simulink model "TailSitter_waypoints_continuous"  (R2018b)
settings: Solver=VariableStepAuto  StartTime=0.0  StopTime=400  RelTol=1e-3
values from neighbouring files (symbols this model uses):
  p =     [ds.mat]    (also in vxs.mat)
undefined symbols (not defined in the file or in its folder): quatnormalize
libraries: aerolibutil x18, simulink x6, sharedutil x3, vrlib x2, simulink_extras x2, sharedtransform x1
(part 2 of 4)

== matlab function TailSitter_waypoints_continuous/Torque_FL ==
  data: u_omegaL output; u_omegaR output; u_deltaL output; u_deltaR output; tao input; states input; u_jointT input; p parameter
function [u_omegaL,u_omegaR, u_deltaL,u_deltaR]  = FL_torques(tao, states, u_jointT, p)


wxr = tao(1); % I wonder if this comversion from omega to tao is right? Depends on Emil Fresk implementation
wyr = tao(2);
wzr = tao(3);
v = states(1:3);
vx = v(1);
vy = v(2);
vz = v(3);
w = states(4:6);
wx = w(1);
wy = w(2);
wz = w(3);
q = states(7:10); % Possibly not needed?
q0=q(1);
q1=q(2);
q2=q(3);
q3=(4);
deltaL = states(11);
deltaR = states(12);
omegaL = states(13);
omegaR = states(14);

% init output vector
u_deltaL = 0;
u_deltaR = 0;
u_omegaL = 0;
u_omegaR = 0;

% If you know of a better way (not counting modifying the code below to use
% p.x notation, plese feel welcome to tell me.
%P = struct2cell(p);
%Pn = fieldnames(p);
%for i=1:numel(P)
%    eval(Pn{i}+"="+string(P{i})+";")
%end
Ts=p.Ts;
m=p.m;
Ix=p.Ix;
Iy=p.Iy;
Iz=p.Iz;
I=p.I;
g=p.g;
rho=p.rho;
propd=p.propd;
K_T=p.K_T;
K_v=p.K_v;
b_w=p.b_w;
Sa=p.Sa;
Saw=p.Saw;
CLdelta=p.CLdelta;
CDdelta=p.CDdelta;
SW=p.SW;
Sw_w=p.Sw_w;
Sw=p.Sw;
b=p.b;
Cmyl=p.Cmyl;
Cwy=p.Cwy;
yf=p.yf;
yt=p.yt;
xW=p.xW;
xf=p.xf;
xac=p.xac;
zW=p.zW;
yw=p.yw;
yW=p.yW;
yWE=p.yWE;
yWEE=p.yWEE;
K_omegaL=p.K_omegaL;
K_omegaR=p.K_omegaR;
K_deltaL=p.K_deltaL;
K_deltaR=p.K_deltaR;
CL_A=p.CL_A;
CL_B=p.CL_B;
CL_C=p.CL_C;
CD_A=p.CD_A;
CD_B=p.CD_B;
CD_C=p.CD_C;
CLB_A=p.CLB_A;
CLB_B=p.CLB_B;
CDB_A=p.CDB_A;
CDB_B=p.CDB_B;
% The constants below are for the polynomial approximations.
% I am lookin into a way of auto-generating them in a struct or something.
a11=p.a11;
a12=p.a12;
a13=p.a13;
a21=p.a21;
a22=p.a22;
a23=p.a23;
a31=p.a31;
a32=p.a32;
a33=p.a33;
a41=p.a41;
a42=p.a42;
a43=p.a43;
b11=p.b11;
b12=p.b12;
b13=p.b13;
b14=p.b14;
b21=p.b21;
b22=p.b22;
b23=p.b23;
b24=p.b24;
b31=p.b31;
b32=p.b32;
b33=p.b33;
b34=p.b34;
c11=p.c11;
c12=p.c12;
c13=p.c13;
c14=p.c14;
c21=p.c21;
c22=p.c22;
c23=p.c23;
c24=p.c24;
c31=p.c31;
c32=p.c32;
c33=p.c33;
c34=p.c34;
c41=p.c41;
c42=p.c42;
c43=p.c43;
c44=p.c44;
% Assuming we made correct choices here it should suffice with this:
%u = [u_deltaA u_jointA u_deltaT]';


% Hey, anyone reading this? Code below is auto-generated because the
% F.L. was just too much of a headache to do
% manyally, so I wrote a script for it.
wn = p.wn;
u_ref =[ ...
                                                                                                                                                                                                                                                                                                                                                                                                                                                                                                                                                                                                                                                                                                                                                                                                                                                                                                                                                                                                                                                                                                                                                                                                                                                                                                                                                                                                                                                                                                                                                                                                                                                                                                                                                                                                                                                                                                                                                                                                                                                                                                                                                                                                                                                                                                                                                                                                                                                                                                                                                                                                                                                                                                                                                                                                                                                                                                                                                                                                                                                                                                                                                                                                                                                                                                                                                                                                                                                                                                                                                                                                                                                                                                                                                                                                                                                                                                                                                                                                                                                                                                                                                                                                                                                                                                                                                                                                                                                                                                                                                                                                                                                                                                                                                                                                                                                                                                                                                                                                                                                                                                                                                                                                                                                                                                                                                                                                                                                                                                                                                                                                                                                                                                                                                                                                                                                                                                                                                                                                                                                                                                                                                                                                                                                                                                                                                                                                                                                                                                                                                                                                                                                                                                                                                                                                                                                                                                                                                                                                                                                                                                                                                                                                                                                                                                                                                                                                                                                                                                                                                                                                                                                                                                                                                                                                                                                                                                                                                                                                                                                                                                                                                                                                                                                                                                                                                                                                                                                                                                                                                                                                                                                                                                                                                                                                                                                                                                                                                                                                                                                                                                                                                                                                                                                                                                                                                                                                                                                                                                                                                                                                                                                                                                                                                                                                                                                                                                                                                                                                                                                                                                                                                                                                                                                                                                                                                                                                                                                                                                                                                                                                                                                                                                                                                                                                                                                                                                                                                                                                                                                                                                                                                                                                                                                                                                                                                                                                                                                                                                                                                                                                                                                                                                                                                                                                                                                                                                                                                                                                                                                                                                                                                                                                                                                                                                                                                                                                                                                                                                                                                                                                                                                                                                                                                                                                                                                                                                                                                                 (4.24e-22*(3.02e112*omegaL^4*wn*abs(omegaL) - 7.01e117*omegaR^3*atan2(1.0*vz, vx) + 1.2e116*omegaL^2*atan2(1.0*vz, vx)*abs(omegaL) - 1.2e116*omegaL^2*atan2(1.0*vz, vx)*abs(omegaR) - 1.2e116*omegaR^2*atan2(1.0*vz, vx)*abs(omegaL) + 1.2e116*omegaR^2*atan2(1.0*vz, vx)*abs(omegaR) + 1.2e116*omegaL^3*atan2(1.0*vz, vx)*sign(omegaL) + 1.2e116*omegaR^3*atan2(1.0*vz, vx)*sign(omegaR) - 4.77e117*omegaL^3*atan2(1.0*vz, vx) + 3.02e112*omegaL^4*wn*abs(omegaR) - 3.02e112*omegaR^4*wn*abs(omegaL) - 3.02e112*omegaR^4*wn*abs(omegaR) + 5.89e117*omegaL^3*wn^2*wx + 5.89e117*omegaR^3*wn^2*wx + 5.89e117*omegaL^3*wn^2*wxr + 5.89e117*omegaR^3*wn^2*wxr - 1.12e117*omegaL^3*wn^2*wy + 1.12e117*omegaR^3*wn^2*wy - 1.12e117*omegaL^3*wn^2*wyr + 1.12e117*omegaR^3*wn^2*wyr - 3.02e112*omegaL^5*wn*sign(omegaL) + 3.02e112*omegaR^5*wn*sign(omegaR) - 7.01e117*omegaL*omegaR^2*atan2(1.0*vz, vx) - 4.77e117*omegaL^2*omegaR*atan2(1.0*vz, vx) - 1.2e116*omegaL^2*wn^2*wz*abs(omegaL) + 1.2e116*omegaL^2*wn^2*wz*abs(omegaR) + 1.2e116*omegaR^2*wn^2*wz*abs(omegaL) - 1.2e116*omegaR^2*wn^2*wz*abs(omegaR) - 1.2e116*omegaL^2*wn^2*wzr*abs(omegaL) + 1.2e116*omegaL^2*wn^2*wzr*abs(omegaR) + 1.2e116*omegaR^2*wn^2*wzr*abs(omegaL) - 1.2e116*omegaR^2*wn^2*wzr*abs(omegaR) - 5.43e117*deltaL*omegaL*omegaR^2*atan2(1.0*vz, vx) - 5.43e117*deltaR*omegaL^2*omegaR*atan2(1.0*vz, vx) + 6.04e112*omegaL^3*omegaR^2*wn*sign(omegaL) - 6.04e112*omegaL^2*omegaR^3*wn*sign(omegaR) - 1.2e116*omegaL^3*wn^2*wz*sign(omegaL) - 1.2e116*omegaR^3*wn^2*wz*sign(omegaR) - 1.2e116*omegaL^3*wn^2*wzr*sign(omegaL) - 1.2e116*omegaR^3*wn^2*wzr*sign(omegaR) - 1.37e114*deltaL*omegaL*omegaR^4*wn + 1.37e114*deltaR*omegaL^4*omegaR*wn + 1.68e119*a11*omegaL^3*wn*wx + 1.68e119*a11*omegaR^3*wn*wx + 1.68e119*b11*omegaL^3*wn*wz + 1.68e119*b11*omegaR^3*wn*wz - 2.89e116*omegaL^3*vx*wn*(vx^2 + vy^2)^(1/2) + 2.89e116*omegaR^3*vx*wn*(vx^2 + vy^2)^(1/2) + 1.16e116*omegaL^3*vx*wn*(vx^2 + vz^2)^(1/2) - 1.71e116*omegaL^3*vy*wn*(vx^2 + vy^2)^(1/2) - 1.16e116*omegaR^3*vx*wn*(vx^2 + vz^2)^(1/2) - 1.71e116*omegaR^3*vy*wn*(vx^2 + vy^2)^(1/2) + 1.19e117*omegaL^3*vz*wn*(vx^2 + vz^2)^(1/2) - 1.19e117*omegaR^3*vz*wn*(vx^2 + vz^2)^(1/2) + 5.8e118*omegaL^3*wn*wy*(vx^2 + vz^2)^(1/2) - 5.8e118*omegaR^3*wn*wy*(vx^2 + vz^2)^(1/2) - 1.2e116*omegaL*omegaR^2*atan2(1.0*vz, vx)*sign(omegaL) - 1.2e116*omegaL^2*omegaR*atan2(1.0*vz, vx)*sign(omegaR) - 1.37e114*deltaL*omegaL^2*omegaR^3*wn + 1.37e114*deltaR*omegaL^3*omegaR^2*wn - 1.02e121*omegaL*vx^2*atan2(1.0*vz, vx)*sign(vx) - 1.02e121*omegaR*vx^2*atan2(1.0*vz, vx)*sign(vx) - 1.02e121*omegaL*vy^2*atan2(1.0*vz, vx)*sign(vx) - 1.02e121*omegaR*vy^2*atan2(1.0*vz, vx)*sign(vx) - 1.02e121*omegaL*vz^2*atan2(1.0*vz, vx)*sign(vx) - 1.02e121*omegaR*vz^2*atan2(1.0*vz, vx)*sign(vx) - 6.04e112*omegaL*omegaR^3*wn*abs(omegaL) + 6.04e112*omegaL^3*omegaR*wn*abs(omegaL) - 6.04e112*omegaL*omegaR^3*wn*abs(omegaR) + 6.04e112*omegaL^3*omegaR*wn*abs(omegaR) + 5.89e117*omegaL*omegaR^2*wn^2*wx + 5.89e117*omegaL^2*omegaR*wn^2*wx + 5.89e117*omegaL*omegaR^2*wn^2*wxr + 5.89e117*omegaL^2*omegaR*wn^2*wxr + 1.12e117*omegaL*omegaR^2*wn^2*wy - 1.12e117*omegaL^2*omegaR*wn^2*wy + 1.12e117*omegaL*omegaR^2*wn^2*wyr - 1.12e117*omegaL^2*omegaR*wn^2*wyr - 3.02e112*omegaL*omegaR^4*wn*sign(omegaL) + 3.02e112*omegaL^4*omegaR*wn*sign(omegaR) - 4.72e120*deltaL*omegaL*vx^2*atan2(1.0*vz, vx)*sign(vx) - 4.72e120*deltaR*omegaR*vx^2*atan2(1.0*vz, vx)*sign(vx) - 4.72e120*deltaL*omegaL*vy^2*atan2(1.0*vz, vx)*sign(vx) - 4.72e120*deltaR*omegaR*vy^2*atan2(1.0*vz, vx)*sign(vx) - 4.72e120*deltaL*omegaL*vz^2*atan2(1.0*vz, vx)*sign(vx) - 4.72e120*deltaR*omegaR*vz^2*atan2(1.0*vz, vx)*sign(vx) + 5.43e117*deltaL*omegaL*omegaR^2*wn^2*wz + 5.43e117*deltaR*omegaL^2*omegaR*wn^2*wz + 5.43e117*deltaL*omegaL*omegaR^2*wn^2*wzr + 5.43e117*deltaR*omegaL^2*omegaR*wn^2*wzr - 3.0e117*c11*omegaL^2*wn*wz*abs(omegaL) + 3.0e117*c11*omegaL^2*wn*wz*abs(omegaR) + 3.0e117*c11*omegaR^2*wn*wz*abs(omegaL) - 3.0e117*c11*omegaR^2*wn*wz*abs(omegaR) + 1.68e119*a31*omegaL^3*vx^2*wn*wx + 1.68e119*a31*omegaR^3*vx^2*wn*wx + 1.68e119*a41*omegaL^3*vx^3*wn*wx + 1.68e119*a41*omegaR^3*vx^3*wn*wx + 1.68e119*a13*omegaL^3*vz^2*wn*wx + 1.68e119*a13*omegaR^3*vz^2*wn*wx + 1.68e119*b31*omegaL^3*vx^2*wn*wz + 1.68e119*b31*omegaR^3*vx^2*wn*wz + 1.68e119*b13*omegaL^3*vz^2*wn*wz + 1.68e119*b14*omegaL^3*vz^3*wn*wz + 1.68e119*b13*omegaR^3*vz^2*wn*wz + 1.68e119*b14*omegaR^3*vz^3*wn*wz - 2.75e115*omegaL^2*vy*wn*abs(omegaL)*(vx^2 + vy^2)^(1/2) + 2.75e115*omegaL^2*vy*wn*abs(omegaR)*(vx^2 + vy^2)^(1/2) + 2.75e115*omegaR^2*vy*wn*abs(omegaL)*(vx^2 + vy^2)^(1/2) - 2.75e115*omegaR^2*vy*wn*abs(omegaR)*(vx^2 + vy^2)^(1/2) - 3.0e117*c11*omegaL^3*wn*wz*sign(omegaL) - 3.0e117*c11*omegaR^3*wn*wz*sign(omegaR) - 2.75e115*omegaL^3*vy*wn*sign(omegaL)*(vx^2 + vy^2)^(1/2) - 2.75e115*omegaR^3*vy*wn*sign(omegaR)*(vx^2 + vy^2)^(1/2) - 2.98e119*omegaL*vy^3*wn*sign(vx)*(vx^2 + vy^2)^(1/2) - 2.98e119*omegaR*vy^3*wn*sign(vx)*(vx^2 + vy^2)^(1/2) - 1.03e120*deltaL*omegaL*vx^4*wn*sign(vx)^2 - 1.19e117*deltaL*omegaR^3*vx^2*wn*sign(vx) + 1.19e117*deltaR*omegaL^3*vx^2*wn*sign(vx) - 1.03e120*deltaL*omegaR*vx^4*wn*sign(vx)^2 + 1.03e120*deltaR*omegaL*vx^4*wn*sign(vx)^2 + 1.03e120*deltaR*omegaR*vx^4*wn*sign(vx)^2 - 1.03e120*deltaL*omegaL*vy^4*wn*sign(vx)^2 - 1.19e117*deltaL*omegaR^3*vy^2*wn*sign(vx) + 1.19e117*deltaR*omegaL^3*vy^2*wn*sign(vx) - 1.03e120*deltaL*omegaR*vy^4*wn*sign(vx)^2 + 1.03e120*deltaR*omegaL*vy^4*wn*sign(vx)^2 + 1.03e120*deltaR*omegaR*vy^4*wn*sign(vx)^2 - 1.03e120*deltaL*omegaL*vz^4*wn*sign(vx)^2 - 1.19e117*deltaL*omegaR^3*vz^2*wn*sign(vx) + 1.19e117*deltaR*omegaL^3*vz^2*wn*sign(vx) - 1.03e120*deltaL*omegaR*vz^4*wn*sign(vx)^2 + 1.03e120*deltaR*omegaL*vz^4*wn*sign(vx)^2 + 1.03e120*deltaR*omegaR*vz^4*wn*sign(vx)^2 + 1.2e116*omegaL*omegaR^2*wn^2*wz*sign(omegaL) + 1.2e116*omegaL^2*omegaR*wn^2*wz*sign(omegaR) + 1.2e116*omegaL*omegaR^2*wn^2*wzr*sign(omegaL) + 1.2e116*omegaL^2*omegaR*wn^2*wzr*sign(omegaR) + 2.89e116*omegaL^3*vx*wn*cos(2.0*atan2(1.0*vy, vx))*(vx^2 + vy^2)^(1/2) - 2.89e116*omegaR^3*vx*wn*cos(2.0*atan2(1.0*vy, vx))*(vx^2 + vy^2)^(1/2) + 1.71e116*omegaL^3*vy*wn*cos(2.0*atan2(1.0*vy, vx))*(vx^2 + vy^2)^(1/2) + 1.71e116*omegaR^3*vy*wn*cos(2.0*atan2(1.0*vy, vx))*(vx^2 + vy^2)^(1/2) - 1.16e117*omegaL^3*vz*wn*cos(2.0*atan2(1.0*vz, vx))*(vx^2 + vz^2)^(1/2) + 1.16e117*omegaR^3*vz*wn*cos(2.0*atan2(1.0*vz, vx))*(vx^2 + vz^2)^(1/2) + 1.02e121*omegaL*vx^2*wn^2*wx*sign(vx) + 1.02e121*omegaR*vx^2*wn^2*wx*sign(vx) + 1.02e121*omegaL*vx^2*wn^2*wxr*sign(vx) + 1.02e121*omegaR*vx^2*wn^2*wxr*sign(vx) + 1.02e121*omegaL*vy^2*wn^2*wx*sign(vx) + 1.02e121*omegaR*vy^2*wn^2*wx*sign(vx) + 1.02e121*omegaL*vy^2*wn^2*wxr*sign(vx) + 1.02e121*omegaR*vy^2*wn^2*wxr*sign(vx) + 1.02e121*omegaL*vz^2*wn^2*wx*sign(vx) + 1.02e121*omegaR*vz^2*wn^2*wx*sign(vx) + 1.02e121*omegaL*vz^2*wn^2*wxr*sign(vx) + 1.02e121*omegaR*vz^2*wn^2*wxr*sign(vx) - 1.03e116*omegaL^3*vx*wn*sin(2.0*atan2(1.0*vy, vx))*(vx^2 + vy^2)^(1/2) - 1.03e116*omegaR^3*vx*wn*sin(2.0*atan2(1.0*vy, vx))*(vx^2 + vy^2)^(1/2) + 1.73e116*omegaL^3*vy*wn*sin(2.0*atan2(1.0*vy, vx))*(vx^2 + vy^2)^(1/2) - 1.73e116*omegaR^3*vy*wn*sin(2.0*atan2(1.0*vy, vx))*(vx^2 + vy^2)^(1/2) + 6.96e116*omegaL^3*vx*wn*sin(2.0*atan2(1.0*vz, vx))*(vx^2 + vz^2)^(1/2) - 6.96e116*omegaR^3*vx*wn*sin(2.0*atan2(1.0*vz, vx))*(vx^2 + vz^2)^(1/2) + 1.68e119*a11*omegaL*omegaR^2*wn*wx + 1.68e119*a11*omegaL^2*omegaR*wn*wx + 1.68e119*b11*omegaL*omegaR^2*wn*wz + 1.68e119*b11*omegaL^2*omegaR*wn*wz + 1.68e119*a21*omegaL^3*vx*wn*wx + 1.68e119*a21*omegaR^3*vx*wn*wx + 1.68e119*a12*omegaL^3*vz*wn*wx + 1.68e119*a12*omegaR^3*vz*wn*wx + 1.68e119*b21*omegaL^3*vx*wn*wz + 1.68e119*b21*omegaR^3*vx*wn*wz + 1.68e119*b12*omegaL^3*vz*wn*wz + 1.68e119*b12*omegaR^3*vz*wn*wz + 2.89e116*omegaL*omegaR^2*vx*wn*(vx^2 + vy^2)^(1/2) - 2.89e116*omegaL^2*omegaR*vx*wn*(vx^2 + vy^2)^(1/2) - 1.16e116*omegaL*omegaR^2*vx*wn*(vx^2 + vz^2)^(1/2) - 1.71e116*omegaL*omegaR^2*vy*wn*(vx^2 + vy^2)^(1/2) + 1.16e116*omegaL^2*omegaR*vx*wn*(vx^2 + vz^2)^(1/2) - 1.71e116*omegaL^2*omegaR*vy*wn*(vx^2 + vy^2)^(1/2) - 1.19e117*omegaL*omegaR^2*vz*wn*(vx^2 + vz^2)^(1/2) + 1.19e117*omegaL^2*omegaR*vz*wn*(vx^2 + vz^2)^(1/2) - 5.8e118*omegaL*omegaR^2*wn*wy*(vx^2 + vz^2)^(1/2) + 5.8e118*omegaL^2*omegaR*wn*wy*(vx^2 + vz^2)^(1/2) - 3.0e117*c31*omegaL^2*vx^2*wn*wz*abs(omegaL) + 3.0e117*c31*omegaL^2*vx^2*wn*wz*abs(omegaR) + 3.0e117*c31*omegaR^2*vx^2*wn*wz*abs(omegaL) - 3.0e117*c41*omegaL^2*vx^3*wn*wz*abs(omegaL) - 3.0e117*c31*omegaR^2*vx^2*wn*wz*abs(omegaR) + 3.0e117*c41*omegaL^2*vx^3*wn*wz*abs(omegaR) + 3.0e117*c41*omegaR^2*vx^3*wn*wz*abs(omegaL) - 3.0e117*c41*omegaR^2*vx^3*wn*wz*abs(omegaR) - 3.0e117*c13*omegaL^2*vz^2*wn*wz*abs(omegaL) - 3.0e117*c14*omegaL^2*vz^3*wn*wz*abs(omegaL) + 3.0e117*c13*omegaL^2*vz^2*wn*wz*abs(omegaR) + 3.0e117*c13*omegaR^2*vz^2*wn*wz*abs(omegaL) + 3.0e117*c14*omegaL^2*vz^3*wn*wz*abs(omegaR) + 3.0e117*c14*omegaR^2*vz^3*wn*wz*abs(omegaL) - 3.0e117*c13*omegaR^2*vz^2*wn*wz*abs(omegaR) - 3.0e117*c14*omegaR^2*vz^3*wn*wz*abs(omegaR) + 1.68e119*a33*omegaL^3*vx^2*vz^2*wn*wx + 1.68e119*a33*omegaR^3*vx^2*vz^2*wn*wx + 1.68e119*a43*omegaL^3*vx^3*vz^2*wn*wx + 1.68e119*a43*omegaR^3*vx^3*vz^2*wn*wx + 1.68e119*b33*omegaL^3*vx^2*vz^2*wn*wz + 1.68e119*b34*omegaL^3*vx^2*vz^3*wn*wz + 1.68e119*b33*omegaR^3*vx^2*vz^2*wn*wz + 1.68e119*b34*omegaR^3*vx^2*vz^3*wn*wz - 3.0e117*c31*omegaL^3*vx^2*wn*wz*sign(omegaL) - 3.0e117*c41*omegaL^3*vx^3*wn*wz*sign(omegaL) - 3.0e117*c31*omegaR^3*vx^2*wn*wz*sign(omegaR) - 3.0e117*c41*omegaR^3*vx^3*wn*wz*sign(omegaR) - 3.0e117*c13*omegaL^3*vz^2*wn*wz*sign(omegaL) - 3.0e117*c14*omegaL^3*vz^3*wn*wz*sign(omegaL) - 3.0e117*c13*omegaR^3*vz^2*wn*wz*sign(omegaR) - 3.0e117*c14*omegaR^3*vz^3*wn*wz*sign(omegaR) - 2.37e117*deltaL*omegaL*omegaR^2*vx^2*wn*sign(vx) - 1.19e117*deltaL*omegaL^2*omegaR*vx^2*wn*sign(vx) + 1.19e117*deltaR*omegaL*omegaR^2*vx^2*wn*sign(vx) + 2.37e117*deltaR*omegaL^2*omegaR*vx^2*wn*sign(vx) - 2.37e117*deltaL*omegaL*omegaR^2*vy^2*wn*sign(vx) - 1.19e117*deltaL*omegaL^2*omegaR*vy^2*wn*sign(vx) + 1.19e117*deltaR*omegaL*omegaR^2*vy^2*wn*sign(vx) + 2.37e117*deltaR*omegaL^2*omegaR*vy^2*wn*sign(vx) - 2.37e117*deltaL*omegaL*omegaR^2*vz^2*wn*sign(vx) - 1.19e117*deltaL*omegaL^2*omegaR*vz^2*wn*sign(vx) + 1.19e117*deltaR*omegaL*omegaR^2*vz^2*wn*sign(vx) + 2.37e117*deltaR*omegaL^2*omegaR*vz^2*wn*sign(vx) + 4.72e120*deltaL*omegaL*vx^2*wn^2*wz*sign(vx) + 4.72e120*deltaR*omegaR*vx^2*wn^2*wz*sign(vx) + 4.72e120*deltaL*omegaL*vx^2*wn^2*wzr*sign(vx) + 4.72e120*deltaR*omegaR*vx^2*wn^2*wzr*sign(vx) + 4.72e120*deltaL*omegaL*vy^2*wn^2*wz*sign(vx) + 4.72e120*deltaR*omegaR*vy^2*wn^2*wz*sign(vx) + 4.72e120*deltaL*omegaL*vy^2*wn^2*wzr*sign(vx) + 4.72e120*deltaR*omegaR*vy^2*wn^2*wzr*sign(vx) + 4.72e120*deltaL*omegaL*vz^2*wn^2*wz*sign(vx) + 4.72e120*deltaR*omegaR*vz^2*wn^2*wz*sign(vx) + 4.72e120*deltaL*omegaL*vz^2*wn^2*wzr*sign(vx) + 4.72e120*deltaR*omegaR*vz^2*wn^2*wzr*sign(vx) - 2.89e116*omegaL*omegaR^2*vx*wn*cos(2.0*atan2(1.0*vy, vx))*(vx^2 + vy^2)^(1/2) + 2.89e116*omegaL^2*omegaR*vx*wn*cos(2.0*atan2(1.0*vy, vx))*(vx^2 + vy^2)^(1/2) + 1.71e116*omegaL*omegaR^2*vy*wn*cos(2.0*atan2(1.0*vy, vx))*(vx^2 + vy^2)^(1/2) + 1.71e116*omegaL^2*omegaR*vy*wn*cos(2.0*atan2(1.0*vy, vx))*(vx^2 + vy^2)^(1/2) + 1.16e117*omegaL*omegaR^2*vz*wn*cos(2.0*atan2(1.0*vz, vx))*(vx^2 + vz^2)^(1/2) - 1.16e117*omegaL^2*omegaR*vz*wn*cos(2.0*atan2(1.0*vz, vx))*(vx^2 + vz^2)^(1/2) + 1.36e119*c11*deltaL*omegaL*omegaR^2*wn*wz + 1.36e119*c11*deltaR*omegaL^2*omegaR*wn*wz - 1.03e116*omegaL*omegaR^2*vx*wn*sin(2.0*atan2(1.0*vy, vx))*(vx^2 + vy^2)^(1/2) - 1.03e116*omegaL^2*omegaR*vx*wn*sin(2.0*atan2(1.0*vy, vx))*(vx^2 + vy^2)^(1/2) - 1.73e116*omegaL*omegaR^2*vy*wn*sin(2.0*atan2(1.0*vy, vx))*(vx^2 + vy^2)^(1/2) + 1.73e116*omegaL^2*omegaR*vy*wn*sin(2.0*atan2(1.0*vy, vx))*(vx^2 + vy^2)^(1/2) - 6.96e116*omegaL*omegaR^2*vx*wn*sin(2.0*atan2(1.0*vz, vx))*(vx^2 + vz^2)^(1/2) + 6.96e116*omegaL^2*omegaR*vx*wn*sin(2.0*atan2(1.0*vz, vx))*(vx^2 + vz^2)^(1/2) + 1.25e117*deltaL*omegaL*omegaR^2*vy*wn*(vx^2 + vy^2)^(1/2) + 1.25e117*deltaR*omegaL^2*omegaR*vy*wn*(vx^2 + vy^2)^(1/2) + 1.68e119*a21*omegaL*omegaR^2*vx*wn*wx + 1.68e119*a21*omegaL^2*omegaR*vx*wn*wx + 1.68e119*a12*omegaL*omegaR^2*vz*wn*wx + 1.68e119*a12*omegaL^2*omegaR*vz*wn*wx + 1.68e119*b21*omegaL*omegaR^2*vx*wn*wz + 1.68e119*b21*omegaL^2*omegaR*vx*wn*wz + 1.68e119*b12*omegaL*omegaR^2*vz*wn*wz + 1.68e119*b12*omegaL^2*omegaR*vz*wn*wz + 1.68e119*a22*omegaL^3*vx*vz*wn*wx + 1.68e119*a22*omegaR^3*vx*vz*wn*wx + 1.68e119*b22*omegaL^3*vx*vz*wn*wz + 1.68e119*b22*omegaR^3*vx*vz*wn*wz - 2.06e120*deltaL*omegaL*vx^2*vy^2*wn*sign(vx)^2 - 2.06e120*deltaL*omegaR*vx^2*vy^2*wn*sign(vx)^2 + 2.06e120*deltaR*omegaL*vx^2*vy^2*wn*sign(vx)^2 + 2.06e120*deltaR*omegaR*vx^2*vy^2*wn*sign(vx)^2 - 2.06e120*deltaL*omegaL*vx^2*vz^2*wn*sign(vx)^2 - 2.06e120*deltaL*omegaR*vx^2*vz^2*wn*sign(vx)^2 + 2.06e120*deltaR*omegaL*vx^2*vz^2*wn*sign(vx)^2 + 2.06e120*deltaR*omegaR*vx^2*vz^2*wn*sign(vx)^2 - 2.06e120*deltaL*omegaL*vy^2*vz^2*wn*sign(vx)^2 - 2.06e120*deltaL*omegaR*vy^2*vz^2*wn*sign(vx)^2 + 2.06e120*deltaR*omegaL*vy^2*vz^2*wn*sign(vx)^2 + 2.06e120*deltaR*omegaR*vy^2*vz^2*wn*sign(vx)^2 + 2.75e115*omegaL^2*vy*wn*cos(2.0*atan2(1.0*vy, vx))*abs(omegaL)*(vx^2 + vy^2)^(1/2) - 2.75e115*omegaL^2*vy*wn*cos(2.0*atan2(1.0*vy, vx))*abs(omegaR)*(vx^2 + vy^2)^(1/2) - 2.75e115*omegaR^2*vy*wn*cos(2.0*atan2(1.0*vy, vx))*abs(omegaL)*(vx^2 + vy^2)^(1/2) + 2.75e115*omegaR^2*vy*wn*cos(2.0*atan2(1.0*vy, vx))*abs(omegaR)*(vx^2 + vy^2)^(1/2) - 1.65e115*omegaL^2*vx*wn*sin(2.0*atan2(1.0*vy, vx))*abs(omegaL)*(vx^2 + vy^2)^(1/2) + 1.65e115*omegaL^2*vx*wn*sin(2.0*atan2(1.0*vy, vx))*abs(omegaR)*(vx^2 + vy^2)^(1/2) + 1.65e115*omegaR^2*vx*wn*sin(2.0*atan2(1.0*vy, vx))*abs(omegaL)*(vx^2 + vy^2)^(1/2) - 1.65e115*omegaR^2*vx*wn*sin(2.0*atan2(1.0*vy, vx))*abs(omegaR)*(vx^2 + vy^2)^(1/2) + 2.75e115*omegaL^3*vy*wn*cos(2.0*atan2(1.0*vy, vx))*sign(omegaL)*(vx^2 + vy^2)^(1/2) + 2.75e115*omegaR^3*vy*wn*cos(2.0*atan2(1.0*vy, vx))*sign(omegaR)*(vx^2 + vy^2)^(1/2) + 2.98e119*omegaL*vy^3*wn*cos(2.0*atan2(1.0*vy, vx))*sign(vx)*(vx^2 + vy^2)^(1/2) + 2.98e119*omegaR*vy^3*wn*cos(2.0*atan2(1.0*vy, vx))*sign(vx)*(vx^2 + vy^2)^(1/2) + 1.68e119*a31*omegaL*omegaR^2*vx^2*wn*wx + 1.68e119*a31*omegaL^2*omegaR*vx^2*wn*wx + 1.68e119*a41*omegaL*omegaR^2*vx^3*wn*wx + 1.68e119*a41*omegaL^2*omegaR*vx^3*wn*wx + 1.68e119*a13*omegaL*omegaR^2*vz^2*wn*wx + 1.68e119*a13*omegaL^2*omegaR*vz^2*wn*wx + 1.68e119*b31*omegaL*omegaR^2*vx^2*wn*wz + 1.68e119*b31*omegaL^2*omegaR*vx^2*wn*wz + 1.68e119*b13*omegaL*omegaR^2*vz^2*wn*wz + 1.68e119*b13*omegaL^2*omegaR*vz^2*wn*wz + 1.68e119*b14*omegaL*omegaR^2*vz^3*wn*wz + 1.68e119*b14*omegaL^2*omegaR*vz^3*wn*wz - 3.0e117*c21*omegaL^2*vx*wn*wz*abs(omegaL) + 3.0e117*c21*omegaL^2*vx*wn*wz*abs(omegaR) + 3.0e117*c21*omegaR^2*vx*wn*wz*abs(omegaL) - 3.0e117*c21*omegaR^2*vx*wn*wz*abs(omegaR) - 3.0e117*c12*omegaL^2*vz*wn*wz*abs(omegaL) + 3.0e117*c12*omegaL^2*vz*wn*wz*abs(omegaR) + 3.0e117*c12*omegaR^2*vz*wn*wz*abs(omegaL) - 3.0e117*c12*omegaR^2*vz*wn*wz*abs(omegaR) - 1.65e115*omegaL^3*vx*wn*sin(2.0*atan2(1.0*vy, vx))*sign(omegaL)*(vx^2 + vy^2)^(1/2) - 1.65e115*omegaR^3*vx*wn*sin(2.0*atan2(1.0*vy, vx))*sign(omegaR)*(vx^2 + vy^2)^(1/2) + 1.68e119*a23*omegaL^3*vx*vz^2*wn*wx + 1.68e119*a23*omegaR^3*vx*vz^2*wn*wx + 1.68e119*a32*omegaL^3*vx^2*vz*wn*wx + 1.68e119*a32*omegaR^3*vx^2*vz*wn*wx + 1.68e119*a42*omegaL^3*vx^3*vz*wn*wx + 1.68e119*a42*omegaR^3*vx^3*vz*wn*wx + 1.68e119*b23*omegaL^3*vx*vz^2*wn*wz + 1.68e119*b24*omegaL^3*vx*vz^3*wn*wz + 1.68e119*b23*omegaR^3*vx*vz^2*wn*wz + 1.68e119*b24*omegaR^3*vx*vz^3*wn*wz + 1.68e119*b32*omegaL^3*vx^2*vz*wn*wz + 1.68e119*b32*omegaR^3*vx^2*vz*wn*wz - 1.79e119*omegaL*vx^3*wn*sin(2.0*atan2(1.0*vy, vx))*sign(vx)*(vx^2 + vy^2)^(1/2) - 1.79e119*omegaR*vx^3*wn*sin(2.0*atan2(1.0*vy, vx))*sign(vx)*(vx^2 + vy^2)^(1/2) + 3.0e117*c11*omegaL*omegaR^2*wn*wz*sign(omegaL) + 3.0e117*c11*omegaL^2*omegaR*wn*wz*sign(omegaR) + 1.08e120*deltaL*omegaL*vy^3*wn*sign(vx)*(vx^2 + vy^2)^(1/2) + 1.08e120*deltaR*omegaR*vy^3*wn*sign(vx)*(vx^2 + vy^2)^(1/2) + 2.75e115*omegaL*omegaR^2*vy*wn*sign(omegaL)*(vx^2 + vy^2)^(1/2) + 2.75e115*omegaL^2*omegaR*vy*wn*sign(omegaR)*(vx^2 + vy^2)^(1/2) - 3.0e117*c21*omegaL^3*vx*wn*wz*sign(omegaL) - 3.0e117*c21*omegaR^3*vx*wn*wz*sign(omegaR) - 3.0e117*c12*omegaL^3*vz*wn*wz*sign(omegaL) - 3.0e117*c12*omegaR^3*vz*wn*wz*sign(omegaR) + 2.92e122*a11*omegaL*vx^2*wn*wx*sign(vx) + 2.92e122*a11*omegaR*vx^2*wn*wx*sign(vx) + 2.92e122*a21*omegaL*vx^3*wn*wx*sign(vx) + 2.92e122*a21*omegaR*vx^3*wn*wx*sign(vx) + 2.92e122*a31*omegaL*vx^4*wn*wx*sign(vx) + 2.92e122*a31*omegaR*vx^4*wn*wx*sign(vx) + 2.92e122*a41*omegaL*vx^5*wn*wx*sign(vx) + 2.92e122*a41*omegaR*vx^5*wn*wx*sign(vx) + 2.92e122*a11*omegaL*vy^2*wn*wx*sign(vx) + 2.92e122*a11*omegaR*vy^2*wn*wx*sign(vx) + 2.92e122*a11*omegaL*vz^2*wn*wx*sign(vx) + 2.92e122*a12*omegaL*vz^3*wn*wx*sign(vx) + 2.92e122*a13*omegaL*vz^4*wn*wx*sign(vx) + 2.92e122*a11*omegaR*vz^2*wn*wx*sign(vx) + 2.92e122*a12*omegaR*vz^3*wn*wx*sign(vx) + 2.92e122*a13*omegaR*vz^4*wn*wx*sign(vx) + 2.92e122*b11*omegaL*vx^2*wn*wz*sign(vx) + 2.92e122*b11*omegaR*vx^2*wn*wz*sign(vx) + 2.92e122*b21*omegaL*vx^3*wn*wz*sign(vx) + 2.92e122*b21*omegaR*vx^3*wn*wz*sign(vx) + 2.92e122*b31*omegaL*vx^4*wn*wz*sign(vx) + 2.92e122*b31*omegaR*vx^4*wn*wz*sign(vx) + 2.92e122*b11*omegaL*vy^2*wn*wz*sign(vx) + 2.92e122*b11*omegaR*vy^2*wn*wz*sign(vx) + 2.92e122*b11*omegaL*vz^2*wn*wz*sign(vx) + 2.92e122*b12*omegaL*vz^3*wn*wz*sign(vx) + 2.92e122*b13*omegaL*vz^4*wn*wz*sign(vx) + 2.92e122*b11*omegaR*vz^2*wn*wz*sign(vx) + 2.92e122*b14*omegaL*vz^5*wn*wz*sign(vx) + 2.92e122*b12*omegaR*vz^3*wn*wz*sign(vx) + 2.92e122*b13*omegaR*vz^4*wn*wz*sign(vx) + 2.92e122*b14*omegaR*vz^5*wn*wz*sign(vx) - 2.98e119*omegaL*vx^2*vy*wn*sign(vx)*(vx^2 + vy^2)^(1/2) - 2.98e119*omegaR*vx^2*vy*wn*sign(vx)*(vx^2 + vy^2)^(1/2) - 2.98e119*omegaL*vy*vz^2*wn*sign(vx)*(vx^2 + vy^2)^(1/2) - 2.98e119*omegaR*vy*vz^2*wn*sign(vx)*(vx^2 + vy^2)^(1/2) - 3.0e117*c33*omegaL^3*vx^2*vz^2*wn*wz*sign(omegaL) - 3.0e117*c34*omegaL^3*vx^2*vz^3*wn*wz*sign(omegaL) - 3.0e117*c43*omegaL^3*vx^3*vz^2*wn*wz*sign(omegaL) - 3.0e117*c33*omegaR^3*vx^2*vz^2*wn*wz*sign(omegaR) - 3.0e117*c44*omegaL^3*vx^3*vz^3*wn*wz*sign(omegaL) - 3.0e117*c34*omegaR^3*vx^2*vz^3*wn*wz*sign(omegaR) - 3.0e117*c43*omegaR^3*vx^3*vz^2*wn*wz*sign(omegaR) - 3.0e117*c44*omegaR^3*vx^3*vz^3*wn*wz*sign(omegaR) - 1.08e120*deltaL*omegaL*vy^3*wn*cos(2.0*atan2(1.0*vy, vx))*sign(vx)*(vx^2 + vy^2)^(1/2) - 1.08e120*deltaR*omegaR*vy^3*wn*cos(2.0*atan2(1.0*vy, vx))*sign(vx)*(vx^2 + vy^2)^(1/2) - 2.75e115*omegaL*omegaR^2*vy*wn*cos(2.0*atan2(1.0*vy, vx))*sign(omegaL)*(vx^2 + vy^2)^(1/2) - 2.75e115*omegaL^2*omegaR*vy*wn*cos(2.0*atan2(1.0*vy, vx))*sign(omegaR)*(vx^2 + vy^2)^(1/2) + 1.36e119*c31*deltaL*omegaL*omegaR^2*vx^2*wn*wz + 1.36e119*c31*deltaR*omegaL^2*omegaR*vx^2*wn*wz + 1.36e119*c41*deltaL*omegaL*omegaR^2*vx^3*wn*wz + 1.36e119*c41*deltaR*omegaL^2*omegaR*vx^3*wn*wz + 1.36e119*c13*deltaL*omegaL*omegaR^2*vz^2*wn*wz + 1.36e119*c14*deltaL*omegaL*omegaR^2*vz^3*wn*wz + 1.36e119*c13*deltaR*omegaL^2*omegaR*vz^2*wn*wz + 1.36e119*c14*deltaR*omegaL^2*omegaR*vz^3*wn*wz + 6.49e119*deltaL*omegaL*vx^3*wn*sin(2.0*atan2(1.0*vy, vx))*sign(vx)*(vx^2 + vy^2)^(1/2) + 6.49e119*deltaR*omegaR*vx^3*wn*sin(2.0*atan2(1.0*vy, vx))*sign(vx)*(vx^2 + vy^2)^(1/2) + 2.98e119*omegaL*vx^2*vy*wn*cos(2.0*atan2(1.0*vy, vx))*sign(vx)*(vx^2 + vy^2)^(1/2) + 2.98e119*omegaR*vx^2*vy*wn*cos(2.0*atan2(1.0*vy, vx))*sign(vx)*(vx^2 + vy^2)^(1/2) + 2.98e119*omegaL*vy*vz^2*wn*cos(2.0*atan2(1.0*vy, vx))*sign(vx)*(vx^2 + vy^2)^(1/2) + 2.98e119*omegaR*vy*vz^2*wn*cos(2.0*atan2(1.0*vy, vx))*sign(vx)*(vx^2 + vy^2)^(1/2) + 1.65e115*omegaL*omegaR^2*vx*wn*sin(2.0*atan2(1.0*vy, vx))*sign(omegaL)*(vx^2 + vy^2)^(1/2) + 1.65e115*omegaL^2*omegaR*vx*wn*sin(2.0*atan2(1.0*vy, vx))*sign(omegaR)*(vx^2 + vy^2)^(1/2) + 1.68e119*a23*omegaL*omegaR^2*vx*vz^2*wn*wx + 1.68e119*a23*omegaL^2*omegaR*vx*vz^2*wn*wx + 1.68e119*a32*omegaL*omegaR^2*vx^2*vz*wn*wx + 1.68e119*a32*omegaL^2*omegaR*vx^2*vz*wn*wx + 1.68e119*a42*omegaL*omegaR^2*vx^3*vz*wn*wx + 1.68e119*a42*omegaL^2*omegaR*vx^3*vz*wn*wx + 1.68e119*b23*omegaL*omegaR^2*vx*vz^2*wn*wz + 1.68e119*b23*omegaL^2*omegaR*vx*vz^2*wn*wz + 1.68e119*b24*omegaL*omegaR^2*vx*vz^3*wn*wz + 1.68e119*b24*omegaL^2*omegaR*vx*vz^3*wn*wz + 1.68e119*b32*omegaL*omegaR^2*vx^2*vz*wn*wz + 1.68e119*b32*omegaL^2*omegaR*vx^2*vz*wn*wz - 3.0e117*c22*omegaL^2*vx*vz*wn*wz*abs(omegaL) + 3.0e117*c22*omegaL^2*vx*vz*wn*wz*abs(omegaR) + 3.0e117*c22*omegaR^2*vx*vz*wn*wz*abs(omegaL) - 3.0e117*c22*omegaR^2*vx*vz*wn*wz*abs(omegaR) + 1.18e122*c11*deltaL*omegaL*vx^2*wn*wz*sign(vx) + 1.18e122*c21*deltaL*omegaL*vx^3*wn*wz*sign(vx) + 1.18e122*c11*deltaR*omegaR*vx^2*wn*wz*sign(vx) + 1.18e122*c31*deltaL*omegaL*vx^4*wn*wz*sign(vx) + 1.18e122*c21*deltaR*omegaR*vx^3*wn*wz*sign(vx) + 1.18e122*c41*deltaL*omegaL*vx^5*wn*wz*sign(vx) + 1.18e122*c31*deltaR*omegaR*vx^4*wn*wz*sign(vx) + 1.18e122*c41*deltaR*omegaR*vx^5*wn*wz*sign(vx) + 1.18e122*c11*deltaL*omegaL*vy^2*wn*wz*sign(vx) + 1.18e122*c11*deltaR*omegaR*vy^2*wn*wz*sign(vx) + 1.18e122*c11*deltaL*omegaL*vz^2*wn*wz*sign(vx) + 1.18e122*c12*deltaL*omegaL*vz^3*wn*wz*sign(vx) + 1.18e122*c13*deltaL*omegaL*vz^4*wn*wz*sign(vx) + 1.18e122*c14*deltaL*omegaL*vz^5*wn*wz*sign(vx) + 1.18e122*c11*deltaR*omegaR*vz^2*wn*wz*sign(vx) + 1.18e122*c12*deltaR*omegaR*vz^3*wn*wz*sign(vx) + 1.18e122*c13*deltaR*omegaR*vz^4*wn*wz*sign(vx) + 1.18e122*c14*deltaR*omegaR*vz^5*wn*wz*sign(vx) - 1.79e119*omegaL*vx*vy^2*wn*sin(2.0*atan2(1.0*vy, vx))*sign(vx)*(vx^2 + vy^2)^(1/2) - 1.79e119*omegaR*vx*vy^2*wn*sin(2.0*atan2(1.0*vy, vx))*sign(vx)*(vx^2 + vy^2)^(1/2) - 1.79e119*omegaL*vx*vz^2*wn*sin(2.0*atan2(1.0*vy, vx))*sign(vx)*(vx^2 + vy^2)^(1/2) - 1.79e119*omegaR*vx*vz^2*wn*sin(2.0*atan2(1.0*vy, vx))*sign(vx)*(vx^2 + vy^2)^(1/2) + 3.0e117*c21*omegaL*omegaR^2*vx*wn*wz*sign(omegaL) + 3.0e117*c21*omegaL^2*omegaR*vx*wn*wz*sign(omegaR) + 3.0e117*c12*omegaL*omegaR^2*vz*wn*wz*sign(omegaL) + 3.0e117*c12*omegaL^2*omegaR*vz*wn*wz*sign(omegaR) + 1.08e120*deltaL*omegaL*vx^2*vy*wn*sign(vx)*(vx^2 + vy^2)^(1/2) + 1.08e120*deltaR*omegaR*vx^2*vy*wn*sign(vx)*(vx^2 + vy^2)^(1/2) + 1.08e120*deltaL*omegaL*vy*vz^2*wn*sign(vx)*(vx^2 + vy^2)^(1/2) + 1.08e120*deltaR*omegaR*vy*vz^2*wn*sign(vx)*(vx^2 + vy^2)^(1/2) - 3.0e117*c22*omegaL^3*vx*vz*wn*wz*sign(omegaL) - 3.0e117*c22*omegaR^3*vx*vz*wn*wz*sign(omegaR) + 2.92e122*a21*omegaL*vx*vy^2*wn*wx*sign(vx) + 2.92e122*a21*omegaR*vx*vy^2*wn*wx*sign(vx) + 2.92e122*a12*omegaL*vx^2*vz*wn*wx*sign(vx) + 2.92e122*a12*omegaR*vx^2*vz*wn*wx*sign(vx) + 2.92e122*a21*omegaL*vx*vz^2*wn*wx*sign(vx) + 2.92e122*a22*omegaL*vx*vz^3*wn*wx*sign(vx) + 2.92e122*a22*omegaL*vx^3*vz*wn*wx*sign(vx) + 2.92e122*a23*omegaL*vx*vz^4*wn*wx*sign(vx) + 2.92e122*a21*omegaR*vx*vz^2*wn*wx*sign(vx) + 2.92e122*a22*omegaR*vx*vz^3*wn*wx*sign(vx) + 2.92e122*a22*omegaR*vx^3*vz*wn*wx*sign(vx) + 2.92e122*a23*omegaR*vx*vz^4*wn*wx*sign(vx) + 2.92e122*a32*omegaL*vx^4*vz*wn*wx*sign(vx) + 2.92e122*a32*omegaR*vx^4*vz*wn*wx*sign(vx) + 2.92e122*a42*omegaL*vx^5*vz*wn*wx*sign(vx) + 2.92e122*a42*omegaR*vx^5*vz*wn*wx*sign(vx) + 2.92e122*a12*omegaL*vy^2*vz*wn*wx*sign(vx) + 2.92e122*a12*omegaR*vy^2*vz*wn*wx*sign(vx) + 2.92e122*b21*omegaL*vx*vy^2*wn*wz*sign(vx) + 2.92e122*b21*omegaR*vx*vy^2*wn*wz*sign(vx) + 2.92e122*b12*omegaL*vx^2*vz*wn*wz*sign(vx) + 2.92e122*b12*omegaR*vx^2*vz*wn*wz*sign(vx) + 2.92e122*b21*omegaL*vx*vz^2*wn*wz*sign(vx) + 2.92e122*b22*omegaL*vx*vz^3*wn*wz*sign(vx) + 2.92e122*b22*omegaL*vx^3*vz*wn*wz*sign(vx) + 2.92e122*b23*omegaL*vx*vz^4*wn*wz*sign(vx) + 2.92e122*b21*omegaR*vx*vz^2*wn*wz*sign(vx) + 2.92e122*b24*omegaL*vx*vz^5*wn*wz*sign(vx) + 2.92e122*b22*omegaR*vx*vz^3*wn*wz*sign(vx) + 2.92e122*b22*omegaR*vx^3*vz*wn*wz*sign(vx) + 2.92e122*b23*omegaR*vx*vz^4*wn*wz*sign(vx) + 2.92e122*b24*omegaR*vx*vz^5*wn*wz*sign(vx) + 2.92e122*b32*omegaL*vx^4*vz*wn*wz*sign(vx) + 2.92e122*b32*omegaR*vx^4*vz*wn*wz*sign(vx) + 2.92e122*b12*omegaL*vy^2*vz*wn*wz*sign(vx) + 2.92e122*b12*omegaR*vy^2*vz*wn*wz*sign(vx) + 1.68e119*a33*omegaL*omegaR^2*vx^2*vz^2*wn*wx + 1.68e119*a33*omegaL^2*omegaR*vx^2*vz^2*wn*wx + 1.68e119*a43*omegaL*omegaR^2*vx^3*vz^2*wn*wx + 1.68e119*a43*omegaL^2*omegaR*vx^3*vz^2*wn*wx + 1.68e119*b33*omegaL*omegaR^2*vx^2*vz^2*wn*wz + 1.68e119*b33*omegaL^2*omegaR*vx^2*vz^2*wn*wz + 1.68e119*b34*omegaL*omegaR^2*vx^2*vz^3*wn*wz + 1.68e119*b34*omegaL^2*omegaR*vx^2*vz^3*wn*wz - 3.0e117*c23*omegaL^2*vx*vz^2*wn*wz*abs(omegaL) - 3.0e117*c24*omegaL^2*vx*vz^3*wn*wz*abs(omegaL) + 3.0e117*c23*omegaL^2*vx*vz^2*wn*wz*abs(omegaR) + 3.0e117*c23*omegaR^2*vx*vz^2*wn*wz*abs(omegaL) + 3.0e117*c24*omegaL^2*vx*vz^3*wn*wz*abs(omegaR) + 3.0e117*c24*omegaR^2*vx*vz^3*wn*wz*abs(omegaL) - 3.0e117*c32*omegaL^2*vx^2*vz*wn*wz*abs(omegaL) - 3.0e117*c23*omegaR^2*vx*vz^2*wn*wz*abs(omegaR) - 3.0e117*c24*omegaR^2*vx*vz^3*wn*wz*abs(omegaR) + 3.0e117*c32*omegaL^2*vx^2*vz*wn*wz*abs(omegaR) + 3.0e117*c32*omegaR^2*vx^2*vz*wn*wz*abs(omegaL) - 3.0e117*c42*omegaL^2*vx^3*vz*wn*wz*abs(omegaL) - 3.0e117*c32*omegaR^2*vx^2*vz*wn*wz*abs(omegaR) + 3.0e117*c42*omegaL^2*vx^3*vz*wn*wz*abs(omegaR) + 3.0e117*c42*omegaR^2*vx^3*vz*wn*wz*abs(omegaL) - 3.0e117*c42*omegaR^2*vx^3*vz*wn*wz*abs(omegaR) + 3.0e117*c31*omegaL*omegaR^2*vx^2*wn*wz*sign(omegaL) + 3.0e117*c31*omegaL^2*omegaR*vx^2*wn*wz*sign(omegaR) + 3.0e117*c41*omegaL*omegaR^2*vx^3*wn*wz*sign(omegaL) + 3.0e117*c41*omegaL^2*omegaR*vx^3*wn*wz*sign(omegaR) + 3.0e117*c13*omegaL*omegaR^2*vz^2*wn*wz*sign(omegaL) + 3.0e117*c14*omegaL*omegaR^2*vz^3*wn*wz*sign(omegaL) + 3.0e117*c13*omegaL^2*omegaR*vz^2*wn*wz*sign(omegaR) + 3.0e117*c14*omegaL^2*omegaR*vz^3*wn*wz*sign(omegaR) - 1.25e117*deltaL*omegaL*omegaR^2*vy*wn*cos(2.0*atan2(1.0*vy, vx))*(vx^2 + vy^2)^(1/2) - 1.25e117*deltaR*omegaL^2*omegaR*vy*wn*cos(2.0*atan2(1.0*vy, vx))*(vx^2 + vy^2)^(1/2) - 3.0e117*c23*omegaL^3*vx*vz^2*wn*wz*sign(omegaL) - 3.0e117*c24*omegaL^3*vx*vz^3*wn*wz*sign(omegaL) - 3.0e117*c32*omegaL^3*vx^2*vz*wn*wz*sign(omegaL) - 3.0e117*c23*omegaR^3*vx*vz^2*wn*wz*sign(omegaR) - 3.0e117*c24*omegaR^3*vx*vz^3*wn*wz*sign(omegaR) - 3.0e117*c42*omegaL^3*vx^3*vz*wn*wz*sign(omegaL) - 3.0e117*c32*omegaR^3*vx^2*vz*wn*wz*sign(omegaR) - 3.0e117*c42*omegaR^3*vx^3*vz*wn*wz*sign(omegaR) + 2.92e122*a31*omegaL*vx^2*vy^2*wn*wx*sign(vx) + 2.92e122*a31*omegaR*vx^2*vy^2*wn*wx*sign(vx) + 2.92e122*a41*omegaL*vx^3*vy^2*wn*wx*sign(vx) + 2.92e122*a41*omegaR*vx^3*vy^2*wn*wx*sign(vx) + 2.92e122*a13*omegaL*vx^2*vz^2*wn*wx*sign(vx) + 2.92e122*a13*omegaR*vx^2*vz^2*wn*wx*sign(vx) + 2.92e122*a23*omegaL*vx^3*vz^2*wn*wx*sign(vx) + 2.92e122*a23*omegaR*vx^3*vz^2*wn*wx*sign(vx) + 2.92e122*a31*omegaL*vx^2*vz^2*wn*wx*sign(vx) + 2.92e122*a32*omegaL*vx^2*vz^3*wn*wx*sign(vx) + 2.92e122*a33*omegaL*vx^2*vz^4*wn*wx*sign(vx) + 2.92e122*a33*omegaL*vx^4*vz^2*wn*wx*sign(vx) + 2.92e122*a31*omegaR*vx^2*vz^2*wn*wx*sign(vx) + 2.92e122*a32*omegaR*vx^2*vz^3*wn*wx*sign(vx) + 2.92e122*a33*omegaR*vx^2*vz^4*wn*wx*sign(vx) + 2.92e122*a33*omegaR*vx^4*vz^2*wn*wx*sign(vx) + 2.92e122*a41*omegaL*vx^3*vz^2*wn*wx*sign(vx) + 2.92e122*a42*omegaL*vx^3*vz^3*wn*wx*sign(vx) + 2.92e122*a43*omegaL*vx^3*vz^4*wn*wx*sign(vx) + 2.92e122*a43*omegaL*vx^5*vz^2*wn*wx*sign(vx) + 2.92e122*a41*omegaR*vx^3*vz^2*wn*wx*sign(vx) + 2.92e122*a42*omegaR*vx^3*vz^3*wn*wx*sign(vx) + 2.92e122*a43*omegaR*vx^3*vz^4*wn*wx*sign(vx) + 2.92e122*a43*omegaR*vx^5*vz^2*wn*wx*sign(vx) + 2.92e122*a13*omegaL*vy^2*vz^2*wn*wx*sign(vx) + 2.92e122*a13*omegaR*vy^2*vz^2*wn*wx*sign(vx) + 2.92e122*b31*omegaL*vx^2*vy^2*wn*wz*sign(vx) + 2.92e122*b31*omegaR*vx^2*vy^2*wn*wz*sign(vx) + 2.92e122*b13*omegaL*vx^2*vz^2*wn*wz*sign(vx) + 2.92e122*b14*omegaL*vx^2*vz^3*wn*wz*sign(vx) + 2.92e122*b13*omegaR*vx^2*vz^2*wn*wz*sign(vx) + 2.92e122*b14*omegaR*vx^2*vz^3*wn*wz*sign(vx) + 2.92e122*b23*omegaL*vx^3*vz^2*wn*wz*sign(vx) + 2.92e122*b24*omegaL*vx^3*vz^3*wn*wz*sign(vx) + 2.92e122*b23*omegaR*vx^3*vz^2*wn*wz*sign(vx) + 2.92e122*b31*omegaL*vx^2*vz^2*wn*wz*sign(vx) + 2.92e122*b24*omegaR*vx^3*vz^3*wn*wz*sign(vx) + 2.92e122*b32*omegaL*vx^2*vz^3*wn*wz*sign(vx) + 2.92e122*b33*omegaL*vx^2*vz^4*wn*wz*sign(vx) + 2.92e122*b33*omegaL*vx^4*vz^2*wn*wz*sign(vx) + 2.92e122*b31*omegaR*vx^2*vz^2*wn*wz*sign(vx) + 2.92e122*b34*omegaL*vx^2*vz^5*wn*wz*sign(vx) + 2.92e122*b34*omegaL*vx^4*vz^3*wn*wz*sign(vx) + 2.92e122*b32*omegaR*vx^2*vz^3*wn*wz*sign(vx) + 2.92e122*b33*omegaR*vx^2*vz^4*wn*wz*sign(vx) + 2.92e122*b33*omegaR*vx^4*vz^2*wn*wz*sign(vx) + 2.92e122*b34*omegaR*vx^2*vz^5*wn*wz*sign(vx) + 2.92e122*b34*omegaR*vx^4*vz^3*wn*wz*sign(vx) + 2.92e122*b13*omegaL*vy^2*vz^2*wn*wz*sign(vx) + 2.92e122*b14*omegaL*vy^2*vz^3*wn*wz*sign(vx) + 2.92e122*b13*omegaR*vy^2*vz^2*wn*wz*sign(vx) + 2.92e122*b14*omegaR*vy^2*vz^3*wn*wz*sign(vx) + 7.47e116*deltaL*omegaL*omegaR^2*vx*wn*sin(2.0*atan2(1.0*vy, vx))*(vx^2 + vy^2)^(1/2) + 7.47e116*deltaR*omegaL^2*omegaR*vx*wn*sin(2.0*atan2(1.0*vy, vx))*(vx^2 + vy^2)^(1/2) + 1.36e119*c21*deltaL*omegaL*omegaR^2*vx*wn*wz + 1.36e119*c21*deltaR*omegaL^2*omegaR*vx*wn*wz + 1.36e119*c12*deltaL*omegaL*omegaR^2*vz*wn*wz + 1.36e119*c12*deltaR*omegaL^2*omegaR*vz*wn*wz + 1.68e119*a22*omegaL*omegaR^2*vx*vz*wn*wx + 1.68e119*a22*omegaL^2*omegaR*vx*vz*wn*wx + 1.68e119*b22*omegaL*omegaR^2*vx*vz*wn*wz + 1.68e119*b22*omegaL^2*omegaR*vx*vz*wn*wz - 3.0e117*c33*omegaL^2*vx^2*vz^2*wn*wz*abs(omegaL) - 3.0e117*c34*omegaL^2*vx^2*vz^3*wn*wz*abs(omegaL) + 3.0e117*c33*omegaL^2*vx^2*vz^2*wn*wz*abs(omegaR) + 3.0e117*c33*omegaR^2*vx^2*vz^2*wn*wz*abs(omegaL) + 3.0e117*c34*omegaL^2*vx^2*vz^3*wn*wz*abs(omegaR) + 3.0e117*c34*omegaR^2*vx^2*vz^3*wn*wz*abs(omegaL) - 3.0e117*c43*omegaL^2*vx^3*vz^2*wn*wz*abs(omegaL) - 3.0e117*c33*omegaR^2*vx^2*vz^2*wn*wz*abs(omegaR) - 3.0e117*c44*omegaL^2*vx^3*vz^3*wn*wz*abs(omegaL) - 3.0e117*c34*omegaR^2*vx^2*vz^3*wn*wz*abs(omegaR) + 3.0e117*c43*omegaL^2*vx^3*vz^2*wn*wz*abs(omegaR) + 3.0e117*c43*omegaR^2*vx^3*vz^2*wn*wz*abs(omegaL) + 3.0e117*c44*omegaL^2*vx^3*vz^3*wn*wz*abs(omegaR) + 3.0e117*c44*omegaR^2*vx^3*vz^3*wn*wz*abs(omegaL) - 3.0e117*c43*omegaR^2*vx^3*vz^2*wn*wz*abs(omegaR) - 3.0e117*c44*omegaR^2*vx^3*vz^3*wn*wz*abs(omegaR) + 1.18e122*c31*deltaL*omegaL*vx^2*vy^2*wn*wz*sign(vx) + 1.18e122*c41*deltaL*omegaL*vx^3*vy^2*wn*wz*sign(vx) + 1.18e122*c31*deltaR*omegaR*vx^2*vy^2*wn*wz*sign(vx) + 1.18e122*c41*deltaR*omegaR*vx^3*vy^2*wn*wz*sign(vx) + 1.18e122*c13*deltaL*omegaL*vx^2*vz^2*wn*wz*sign(vx) + 1.18e122*c14*deltaL*omegaL*vx^2*vz^3*wn*wz*sign(vx) + 1.18e122*c23*deltaL*omegaL*vx^3*vz^2*wn*wz*sign(vx) + 1.18e122*c13*deltaR*omegaR*vx^2*vz^2*wn*wz*sign(vx) + 1.18e122*c24*deltaL*omegaL*vx^3*vz^3*wn*wz*sign(vx) + 1.18e122*c14*deltaR*omegaR*vx^2*vz^3*wn*wz*sign(vx) + 1.18e122*c31*deltaL*omegaL*vx^2*vz^2*wn*wz*sign(vx) + 1.18e122*c32*deltaL*omegaL*vx^2*vz^3*wn*wz*sign(vx) + 1.18e122*c33*deltaL*omegaL*vx^2*vz^4*wn*wz*sign(vx) + 1.18e122*c33*deltaL*omegaL*vx^4*vz^2*wn*wz*sign(vx) + 1.18e122*c23*deltaR*omegaR*vx^3*vz^2*wn*wz*sign(vx) + 1.18e122*c34*deltaL*omegaL*vx^2*vz^5*wn*wz*sign(vx) + 1.18e122*c34*deltaL*omegaL*vx^4*vz^3*wn*wz*sign(vx) + 1.18e122*c24*deltaR*omegaR*vx^3*vz^3*wn*wz*sign(vx) + 1.18e122*c41*deltaL*omegaL*vx^3*vz^2*wn*wz*sign(vx) + 1.18e122*c31*deltaR*omegaR*vx^2*vz^2*wn*wz*sign(vx) + 1.18e122*c42*deltaL*omegaL*vx^3*vz^3*wn*wz*sign(vx) + 1.18e122*c32*deltaR*omegaR*vx^2*vz^3*wn*wz*sign(vx) + 1.18e122*c43*deltaL*omegaL*vx^3*vz^4*wn*wz*sign(vx) + 1.18e122*c43*deltaL*omegaL*vx^5*vz^2*wn*wz*sign(vx) + 1.18e122*c33*deltaR*omegaR*vx^2*vz^4*wn*wz*sign(vx) + 1.18e122*c33*deltaR*omegaR*vx^4*vz^2*wn*wz*sign(vx) + 1.18e122*c44*deltaL*omegaL*vx^3*vz^5*wn*wz*sign(vx) + 1.18e122*c44*deltaL*omegaL*vx^5*vz^3*wn*wz*sign(vx) + 1.18e122*c34*deltaR*omegaR*vx^2*vz^5*wn*wz*sign(vx) + 1.18e122*c34*deltaR*omegaR*vx^4*vz^3*wn*wz*sign(vx) + 1.18e122*c41*deltaR*omegaR*vx^3*vz^2*wn*wz*sign(vx) + 1.18e122*c42*deltaR*omegaR*vx^3*vz^3*wn*wz*sign(vx) + 1.18e122*c43*deltaR*omegaR*vx^3*vz^4*wn*wz*sign(vx) + 1.18e122*c43*deltaR*omegaR*vx^5*vz^2*wn*wz*sign(vx) + 1.18e122*c44*deltaR*omegaR*vx^3*vz^5*wn*wz*sign(vx) + 1.18e122*c44*deltaR*omegaR*vx^5*vz^3*wn*wz*sign(vx) + 1.18e122*c13*deltaL*omegaL*vy^2*vz^2*wn*wz*sign(vx) + 1.18e122*c14*deltaL*omegaL*vy^2*vz^3*wn*wz*sign(vx) + 1.18e122*c13*deltaR*omegaR*vy^2*vz^2*wn*wz*sign(vx) + 1.18e122*c14*deltaR*omegaR*vy^2*vz^3*wn*wz*sign(vx) + 3.0e117*c23*omegaL*omegaR^2*vx*vz^2*wn*wz*sign(omegaL) + 3.0e117*c24*omegaL*omegaR^2*vx*vz^3*wn*wz*sign(omegaL) + 3.0e117*c23*omegaL^2*omegaR*vx*vz^2*wn*wz*sign(omegaR) + 3.0e117*c24*omegaL^2*omegaR*vx*vz^3*wn*wz*sign(omegaR) + 3.0e117*c32*omegaL*omegaR^2*vx^2*vz*wn*wz*sign(omegaL) + 3.0e117*c32*omegaL^2*omegaR*vx^2*vz*wn*wz*sign(omegaR) + 3.0e117*c42*omegaL*omegaR^2*vx^3*vz*wn*wz*sign(omegaL) + 3.0e117*c42*omegaL^2*omegaR*vx^3*vz*wn*wz*sign(omegaR) + 2.92e122*a23*omegaL*vx*vy^2*vz^2*wn*wx*sign(vx) + 2.92e122*a23*omegaR*vx*vy^2*vz^2*wn*wx*sign(vx) + 2.92e122*a32*omegaL*vx^2*vy^2*vz*wn*wx*sign(vx) + 2.92e122*a32*omegaR*vx^2*vy^2*vz*wn*wx*sign(vx) + 2.92e122*a42*omegaL*vx^3*vy^2*vz*wn*wx*sign(vx) + 2.92e122*a42*omegaR*vx^3*vy^2*vz*wn*wx*sign(vx) + 2.92e122*b23*omegaL*vx*vy^2*vz^2*wn*wz*sign(vx) + 2.92e122*b24*omegaL*vx*vy^2*vz^3*wn*wz*sign(vx) + 2.92e122*b23*omegaR*vx*vy^2*vz^2*wn*wz*sign(vx) + 2.92e122*b24*omegaR*vx*vy^2*vz^3*wn*wz*sign(vx) + 2.92e122*b32*omegaL*vx^2*vy^2*vz*wn*wz*sign(vx) + 2.92e122*b32*omegaR*vx^2*vy^2*vz*wn*wz*sign(vx) + 1.36e119*c22*deltaL*omegaL*omegaR^2*vx*vz*wn*wz + 1.36e119*c22*deltaR*omegaL^2*omegaR*vx*vz*wn*wz + 3.0e117*c33*omegaL*omegaR^2*vx^2*vz^2*wn*wz*sign(omegaL) + 3.0e117*c34*omegaL*omegaR^2*vx^2*vz^3*wn*wz*sign(omegaL) + 3.0e117*c33*omegaL^2*omegaR*vx^2*vz^2*wn*wz*sign(omegaR) + 3.0e117*c34*omegaL^2*omegaR*vx^2*vz^3*wn*wz*sign(omegaR) + 3.0e117*c43*omegaL*omegaR^2*vx^3*vz^2*wn*wz*sign(omegaL) + 3.0e117*c44*omegaL*omegaR^2*vx^3*vz^3*wn*wz*sign(omegaL) + 3.0e117*c43*omegaL^2*omegaR*vx^3*vz^2*wn*wz*sign(omegaR) + 3.0e117*c44*omegaL^2*omegaR*vx^3*vz^3*wn*wz*sign(omegaR) + 2.92e122*a33*omegaL*vx^2*vy^2*vz^2*wn*wx*sign(vx) + 2.92e122*a33*omegaR*vx^2*vy^2*vz^2*wn*wx*sign(vx) + 2.92e122*a43*omegaL*vx^3*vy^2*vz^2*wn*wx*sign(vx) + 2.92e122*a43*omegaR*vx^3*vy^2*vz^2*wn*wx*sign(vx) + 2.92e122*b33*omegaL*vx^2*vy^2*vz^2*wn*wz*sign(vx) + 2.92e122*b34*omegaL*vx^2*vy^2*vz^3*wn*wz*sign(vx) + 2.92e122*b33*omegaR*vx^2*vy^2*vz^2*wn*wz*sign(vx) + 2.92e122*b34*omegaR*vx^2*vy^2*vz^3*wn*wz*sign(vx) - 1.08e120*deltaL*omegaL*vx^2*vy*wn*cos(2.0*atan2(1.0*vy, vx))*sign(vx)*(vx^2 + vy^2)^(1/2) - 1.08e120*deltaR*omegaR*vx^2*vy*wn*cos(2.0*atan2(1.0*vy, vx))*sign(vx)*(vx^2 + vy^2)^(1/2) - 1.08e120*deltaL*omegaL*vy*vz^2*wn*cos(2.0*atan2(1.0*vy, vx))*sign(vx)*(vx^2 + vy^2)^(1/2) - 1.08e120*deltaR*omegaR*vy*vz^2*wn*cos(2.0*atan2(1.0*vy, vx))*sign(vx)*(vx^2 + vy^2)^(1/2) + 1.36e119*c23*deltaL*omegaL*omegaR^2*vx*vz^2*wn*wz + 1.36e119*c24*deltaL*omegaL*omegaR^2*vx*vz^3*wn*wz + 1.36e119*c23*deltaR*omegaL^2*omegaR*vx*vz^2*wn*wz + 1.36e119*c24*deltaR*omegaL^2*omegaR*vx*vz^3*wn*wz + 1.36e119*c32*deltaL*omegaL*omegaR^2*vx^2*vz*wn*wz + 1.36e119*c32*deltaR*omegaL^2*omegaR*vx^2*vz*wn*wz + 1.36e119*c42*deltaL*omegaL*omegaR^2*vx^3*vz*wn*wz + 1.36e119*c42*deltaR*omegaL^2*omegaR*vx^3*vz*wn*wz + 6.49e119*deltaL*omegaL*vx*vy^2*wn*sin(2.0*atan2(1.0*vy, vx))*sign(vx)*(vx^2 + vy^2)^(1/2) + 6.49e119*deltaR*omegaR*vx*vy^2*wn*sin(2.0*atan2(1.0*vy, vx))*sign(vx)*(vx^2 + vy^2)^(1/2) + 6.49e119*deltaL*omegaL*vx*vz^2*wn*sin(2.0*atan2(1.0*vy, vx))*sign(vx)*(vx^2 + vy^2)^(1/2) + 6.49e119*deltaR*omegaR*vx*vz^2*wn*sin(2.0*atan2(1.0*vy, vx))*sign(vx)*(vx^2 + vy^2)^(1/2) + 1.18e122*c21*deltaL*omegaL*vx*vy^2*wn*wz*sign(vx) + 1.18e122*c21*deltaR*omegaR*vx*vy^2*wn*wz*sign(vx) + 1.18e122*c12*deltaL*omegaL*vx^2*vz*wn*wz*sign(vx) + 1.18e122*c21*deltaL*omegaL*vx*vz^2*wn*wz*sign(vx) + 1.18e122*c22*deltaL*omegaL*vx*vz^3*wn*wz*sign(vx) + 1.18e122*c22*deltaL*omegaL*vx^3*vz*wn*wz*sign(vx) + 1.18e122*c12*deltaR*omegaR*vx^2*vz*wn*wz*sign(vx) + 1.18e122*c23*deltaL*omegaL*vx*vz^4*wn*wz*sign(vx) + 1.18e122*c24*deltaL*omegaL*vx*vz^5*wn*wz*sign(vx) + 1.18e122*c21*deltaR*omegaR*vx*vz^2*wn*wz*sign(vx) + 1.18e122*c32*deltaL*omegaL*vx^4*vz*wn*wz*sign(vx) + 1.18e122*c22*deltaR*omegaR*vx*vz^3*wn*wz*sign(vx) + 1.18e122*c22*deltaR*omegaR*vx^3*vz*wn*wz*sign(vx) + 1.18e122*c23*deltaR*omegaR*vx*vz^4*wn*wz*sign(vx) + 1.18e122*c24*deltaR*omegaR*vx*vz^5*wn*wz*sign(vx) + 1.18e122*c42*deltaL*omegaL*vx^5*vz*wn*wz*sign(vx) + 1.18e122*c32*deltaR*omegaR*vx^4*vz*wn*wz*sign(vx) + 1.18e122*c42*deltaR*omegaR*vx^5*vz*wn*wz*sign(vx) + 1.18e122*c12*deltaL*omegaL*vy^2*vz*wn*wz*sign(vx) + 1.18e122*c12*deltaR*omegaR*vy^2*vz*wn*wz*sign(vx) + 3.0e117*c22*omegaL*omegaR^2*vx*vz*wn*wz*sign(omegaL) + 3.0e117*c22*omegaL^2*omegaR*vx*vz*wn*wz*sign(omegaR) + 2.92e122*a22*omegaL*vx*vy^2*vz*wn*wx*sign(vx) + 2.92e122*a22*omegaR*vx*vy^2*vz*wn*wx*sign(vx) + 2.92e122*b22*omegaL*vx*vy^2*vz*wn*wz*sign(vx) + 2.92e122*b22*omegaR*vx*vy^2*vz*wn*wz*sign(vx) + 1.36e119*c33*deltaL*omegaL*omegaR^2*vx^2*vz^2*wn*wz + 1.36e119*c34*deltaL*omegaL*omegaR^2*vx^2*vz^3*wn*wz + 1.36e119*c33*deltaR*omegaL^2*omegaR*vx^2*vz^2*wn*wz + 1.36e119*c34*deltaR*omegaL^2*omegaR*vx^2*vz^3*wn*wz + 1.36e119*c43*deltaL*omegaL*omegaR^2*vx^3*vz^2*wn*wz + 1.36e119*c44*deltaL*omegaL*omegaR^2*vx^3*vz^3*wn*wz + 1.36e119*c43*deltaR*omegaL^2*omegaR*vx^3*vz^2*wn*wz + 1.36e119*c44*deltaR*omegaL^2*omegaR*vx^3*vz^3*wn*wz + 1.18e122*c22*deltaL*omegaL*vx*vy^2*vz*wn*wz*sign(vx) + 1.18e122*c22*deltaR*omegaR*vx*vy^2*vz*wn*wz*sign(vx) + 1.18e122*c23*deltaL*omegaL*vx*vy^2*vz^2*wn*wz*sign(vx) + 1.18e122*c24*deltaL*omegaL*vx*vy^2*vz^3*wn*wz*sign(vx) + 1.18e122*c32*deltaL*omegaL*vx^2*vy^2*vz*wn*wz*sign(vx) + 1.18e122*c23*deltaR*omegaR*vx*vy^2*vz^2*wn*wz*sign(vx) + 1.18e122*c24*deltaR*omegaR*vx*vy^2*vz^3*wn*wz*sign(vx) + 1.18e122*c42*deltaL*omegaL*vx^3*vy^2*vz*wn*wz*sign(vx) + 1.18e122*c32*deltaR*omegaR*vx^2*vy^2*vz*wn*wz*sign(vx) + 1.18e122*c42*deltaR*omegaR*vx^3*vy^2*vz*wn*wz*sign(vx) + 1.18e122*c33*deltaL*omegaL*vx^2*vy^2*vz^2*wn*wz*sign(vx) + 1.18e122*c34*deltaL*omegaL*vx^2*vy^2*vz^3*wn*wz*sign(vx) + 1.18e122*c43*deltaL*omegaL*vx^3*vy^2*vz^2*wn*wz*sign(vx) + 1.18e122*c33*deltaR*omegaR*vx^2*vy^2*vz^2*wn*wz*sign(vx) + 1.18e122*c44*deltaL*omegaL*vx^3*vy^2*vz^3*wn*wz*sign(vx) + 1.18e122*c34*deltaR*omegaR*vx^2*vy^2*vz^3*wn*wz*sign(vx) + 1.18e122*c43*deltaR*omegaR*vx^3*vy^2*vz^2*wn*wz*sign(vx) + 1.18e122*c44*deltaR*omegaR*vx^3*vy^2*vz^3*wn*wz*sign(vx)))/((omegaL + omegaR)*(2.9e93*omegaL^2*omegaR^2 + 2.52e96*omegaL^2*vx^2*sign(vx) + 2.52e96*omegaL^2*vy^2*sign(vx) + 2.52e96*omegaL^2*vz^2*sign(vx) + 2.52e96*omegaR^2*vx^2*sign(vx) + 2.52e96*omegaR^2*vy^2*sign(vx) + 2.52e96*omegaR^2*vz^2*sign(vx) + 2.19e99*vx^4*sign(vx)^2 + 4.37e99*vx^2*vy^2*sign(vx)^2 + 4.37e99*vx^2*vz^2*sign(vx)^2 + 2.19e99*vy^4*sign(vx)^2 + 4.37e99*vy^2*vz^2*sign(vx)^2 + 2.19e99*vz^4*sign(vx)^2));
 (1.93e-23*(3.32e113*omegaL^4*wn*abs(omegaL) + 7.71e118*omegaR^3*atan2(1.0*vz, vx) + 1.32e117*omegaL^2*atan2(1.0*vz, vx)*abs(omegaL) - 1.32e117*omegaL^2*atan2(1.0*vz, vx)*abs(omegaR) + 1.32e117*omegaR^2*atan2(1.0*vz, vx)*abs(omegaL) - 1.32e117*omegaR^2*atan2(1.0*vz, vx)*abs(omegaR) + 1.32e117*omegaL^3*atan2(1.0*vz, vx)*sign(omegaL) - 1.32e117*omegaR^3*atan2(1.0*vz, vx)*sign(omegaR) - 5.24e118*omegaL^3*atan2(1.0*vz, vx) + 3.32e113*omegaL^4*wn*abs(omegaR) + 3.32e113*omegaR^4*wn*abs(omegaL) + 3.32e113*omegaR^4*wn*abs(omegaR) + 6.47e118*omegaL^3*wn^2*wx - 6.47e118*omegaR^3*wn^2*wx + 6.47e118*omegaL^3*wn^2*wxr - 6.47e118*omegaR^3*wn^2*wxr - 1.23e118*omegaL^3*wn^2*wy - 1.23e118*omegaR^3*wn^2*wy - 1.23e118*omegaL^3*wn^2*wyr - 1.23e118*omegaR^3*wn^2*wyr - 3.32e113*omegaL^5*wn*sign(omegaL) - 3.32e113*omegaR^5*wn*sign(omegaR) + 7.71e118*omegaL*omegaR^2*atan2(1.0*vz, vx) - 5.24e118*omegaL^2*omegaR*atan2(1.0*vz, vx) + 2.29e120*vx^2*atan2(1.0*vz, vx)*abs(omegaL)*sign(vx) - 2.29e120*vx^2*atan2(1.0*vz, vx)*abs(omegaR)*sign(vx) + 2.29e120*vy^2*atan2(1.0*vz, vx)*abs(omegaL)*sign(vx) - 2.29e120*vy^2*atan2(1.0*vz, vx)*abs(omegaR)*sign(vx) + 2.29e120*vz^2*atan2(1.0*vz, vx)*abs(omegaL)*sign(vx) - 2.29e120*vz^2*atan2(1.0*vz, vx)*abs(omegaR)*sign(vx) + 6.64e113*omegaL^2*omegaR^2*wn*abs(omegaL) + 6.64e113*omegaL^2*omegaR^2*wn*abs(omegaR) - 1.32e117*omegaL^2*wn^2*wz*abs(omegaL) + 1.32e117*omegaL^2*wn^2*wz*abs(omegaR) - 1.32e117*omegaR^2*wn^2*wz*abs(omegaL) + 1.32e117*omegaR^2*wn^2*wz*abs(omegaR) - 1.32e117*omegaL^2*wn^2*wzr*abs(omegaL) + 1.32e117*omegaL^2*wn^2*wzr*abs(omegaR) - 1.32e117*omegaR^2*wn^2*wzr*abs(omegaL) + 1.32e117*omegaR^2*wn^2*wzr*abs(omegaR) + 5.97e118*deltaL*omegaL*omegaR^2*atan2(1.0*vz, vx) - 5.97e118*deltaR*omegaL^2*omegaR*atan2(1.0*vz, vx) - 1.32e117*omegaL^3*wn^2*wz*sign(omegaL) + 1.32e117*omegaR^3*wn^2*wz*sign(omegaR) - 1.32e117*omegaL^3*wn^2*wzr*sign(omegaL) + 1.32e117*omegaR^3*wn^2*wzr*sign(omegaR) + 1.5e115*deltaL*omegaL*omegaR^4*wn + 1.5e115*deltaR*omegaL^4*omegaR*wn + 1.85e120*a11*omegaL^3*wn*wx - 1.85e120*a11*omegaR^3*wn*wx + 1.85e120*b11*omegaL^3*wn*wz - 1.85e120*b11*omegaR^3*wn*wz - 3.18e117*omegaL^3*vx*wn*(vx^2 + vy^2)^(1/2) - 3.18e117*omegaR^3*vx*wn*(vx^2 + vy^2)^(1/2) + 1.28e117*omegaL^3*vx*wn*(vx^2 + vz^2)^(1/2) - 1.89e117*omegaL^3*vy*wn*(vx^2 + vy^2)^(1/2) + 1.28e117*omegaR^3*vx*wn*(vx^2 + vz^2)^(1/2) + 1.89e117*omegaR^3*vy*wn*(vx^2 + vy^2)^(1/2) + 1.31e118*omegaL^3*vz*wn*(vx^2 + vz^2)^(1/2) + 1.31e118*omegaR^3*vz*wn*(vx^2 + vz^2)^(1/2) + 6.38e119*omegaL^3*wn*wy*(vx^2 + vz^2)^(1/2) + 6.38e119*omegaR^3*wn*wy*(vx^2 + vz^2)^(1/2) + 1.32e117*omegaL*omegaR^2*atan2(1.0*vz, vx)*sign(omegaL) - 1.32e117*omegaL^2*omegaR*atan2(1.0*vz, vx)*sign(omegaR) + 1.5e115*deltaL*omegaL^2*omegaR^3*wn + 1.5e115*deltaR*omegaL^3*omegaR^2*wn + 2.14e121*omegaL*vx^2*atan2(1.0*vz, vx)*sign(vx) + 2.14e121*omegaR*vx^2*atan2(1.0*vz, vx)*sign(vx) + 2.14e121*omegaL*vy^2*atan2(1.0*vz, vx)*sign(vx) + 2.14e121*omegaR*vy^2*atan2(1.0*vz, vx)*sign(vx) + 2.14e121*omegaL*vz^2*atan2(1.0*vz, vx)*sign(vx) + 2.14e121*omegaR*vz^2*atan2(1.0*vz, vx)*sign(vx) + 6.64e113*omegaL*omegaR^3*wn*abs(omegaL) + 6.64e113*omegaL^3*omegaR*wn*abs(omegaL) + 6.64e113*omegaL*omegaR^3*wn*abs(omegaR) + 6.64e113*omegaL^3*omegaR*wn*abs(omegaR) - 6.47e118*omegaL*omegaR^2*wn^2*wx + 6.47e118*omegaL^2*omegaR*wn^2*wx - 6.47e118*omegaL*omegaR^2*wn^2*wxr + 6.47e118*omegaL^2*omegaR*wn^2*wxr - 1.23e118*omegaL*omegaR^2*wn^2*wy - 1.23e118*omegaL^2*omegaR*wn^2*wy - 1.23e118*omegaL*omegaR^2*wn^2*wyr - 1.23e118*omegaL^2*omegaR*wn^2*wyr + 3.32e113*omegaL*omegaR^4*wn*sign(omegaL) + 3.32e113*omegaL^4*omegaR*wn*sign(omegaR) + 5.77e116*omegaL^2*vx^2*wn*abs(omegaL)*sign(vx) + 5.77e116*omegaL^2*vx^2*wn*abs(omegaR)*sign(vx) + 5.77e116*omegaR^2*vx^2*wn*abs(omegaL)*sign(vx) + 5.77e116*omegaR^2*vx^2*wn*abs(omegaR)*sign(vx) + 5.77e116*omegaL^2*vy^2*wn*abs(omegaL)*sign(vx) + 5.77e116*omegaL^2*vy^2*wn*abs(omegaR)*sign(vx) + 5.77e116*omegaR^2*vy^2*wn*abs(omegaL)*sign(vx) + 5.77e116*omegaR^2*vy^2*wn*abs(omegaR)*sign(vx) + 5.77e116*omegaL^2*vz^2*wn*abs(omegaL)*sign(vx) + 5.77e116*omegaL^2*vz^2*wn*abs(omegaR)*sign(vx) + 5.77e116*omegaR^2*vz^2*wn*abs(omegaL)*sign(vx) + 5.77e116*omegaR^2*vz^2*wn*abs(omegaR)*sign(vx) - 2.29e120*vx^2*wn^2*wz*abs(omegaL)*sign(vx) + 2.29e120*vx^2*wn^2*wz*abs(omegaR)*sign(vx) - 2.29e120*vx^2*wn^2*wzr*abs(omegaL)*sign(vx) + 2.29e120*vx^2*wn^2*wzr*abs(omegaR)*sign(vx) - 2.29e120*vy^2*wn^2*wz*abs(omegaL)*sign(vx) + 2.29e120*vy^2*wn^2*wz*abs(omegaR)*sign(vx) - 2.29e120*vy^2*wn^2*wzr*abs(omegaL)*sign(vx) + 2.29e120*vy^2*wn^2*wzr*abs(omegaR)*sign(vx) - 2.29e120*vz^2*wn^2*wz*abs(omegaL)*sign(vx) + 2.29e120*vz^2*wn^2*wz*abs(omegaR)*sign(vx) - 2.29e120*vz^2*wn^2*wzr*abs(omegaL)*sign(vx) + 2.29e120*vz^2*wn^2*wzr*abs(omegaR)*sign(vx) + 5.19e121*deltaL*omegaL*vx^2*atan2(1.0*vz, vx)*sign(vx) - 5.19e121*deltaR*omegaR*vx^2*atan2(1.0*vz, vx)*sign(vx) + 5.19e121*deltaL*omegaL*vy^2*atan2(1.0*vz, vx)*sign(vx) - 5.19e121*deltaR*omegaR*vy^2*atan2(1.0*vz, vx)*sign(vx) + 5.19e121*deltaL*omegaL*vz^2*atan2(1.0*vz, vx)*sign(vx) - 5.19e121*deltaR*omegaR*vz^2*atan2(1.0*vz, vx)*sign(vx) - 5.77e116*omegaL^3*vx^2*wn*sign(omegaL)*sign(vx) - 5.77e116*omegaR^3*vx^2*wn*sign(omegaR)*sign(vx) - 5.77e116*omegaL^3*vy^2*wn*sign(omegaL)*sign(vx) - 5.77e116*omegaR^3*vy^2*wn*sign(omegaR)*sign(vx) - 5.77e116*omegaL^3*vz^2*wn*sign(omegaL)*sign(vx) - 5.77e116*omegaR^3*vz^2*wn*sign(omegaR)*sign(vx) - 5.97e118*deltaL*omegaL*omegaR^2*wn^2*wz + 5.97e118*deltaR*omegaL^2*omegaR*wn^2*wz - 5.97e118*deltaL*omegaL*omegaR^2*wn^2*wzr + 5.97e118*deltaR*omegaL^2*omegaR*wn^2*wzr - 3.3e118*c11*omegaL^2*wn*wz*abs(omegaL) + 3.3e118*c11*omegaL^2*wn*wz*abs(omegaR) - 3.3e118*c11*omegaR^2*wn*wz*abs(omegaL) + 3.3e118*c11*omegaR^2*wn*wz*abs(omegaR) + 1.85e120*a31*omegaL^3*vx^2*wn*wx - 1.85e120*a31*omegaR^3*vx^2*wn*wx + 1.85e120*a41*omegaL^3*vx^3*wn*wx - 1.85e120*a41*omegaR^3*vx^3*wn*wx + 1.85e120*a13*omegaL^3*vz^2*wn*wx - 1.85e120*a13*omegaR^3*vz^2*wn*wx + 1.85e120*b31*omegaL^3*vx^2*wn*wz - 1.85e120*b31*omegaR^3*vx^2*wn*wz + 1.85e120*b13*omegaL^3*vz^2*wn*wz + 1.85e120*b14*omegaL^3*vz^3*wn*wz - 1.85e120*b13*omegaR^3*vz^2*wn*wz - 1.85e120*b14*omegaR^3*vz^3*wn*wz - 3.03e116*omegaL^2*vy*wn*abs(omegaL)*(vx^2 + vy^2)^(1/2) + 3.03e116*omegaL^2*vy*wn*abs(omegaR)*(vx^2 + vy^2)^(1/2) - 3.03e116*omegaR^2*vy*wn*abs(omegaL)*(vx^2 + vy^2)^(1/2) + 3.03e116*omegaR^2*vy*wn*abs(omegaR)*(vx^2 + vy^2)^(1/2) - 3.3e118*c11*omegaL^3*wn*wz*sign(omegaL) + 3.3e118*c11*omegaR^3*wn*wz*sign(omegaR) - 3.03e116*omegaL^3*vy*wn*sign(omegaL)*(vx^2 + vy^2)^(1/2) + 3.03e116*omegaR^3*vy*wn*sign(omegaR)*(vx^2 + vy^2)^(1/2) - 5.52e120*omegaL*vx^3*wn*sign(vx)*(vx^2 + vy^2)^(1/2) - 5.52e120*omegaR*vx^3*wn*sign(vx)*(vx^2 + vy^2)^(1/2) + 2.22e120*omegaL*vx^3*wn*sign(vx)*(vx^2 + vz^2)^(1/2) + 2.22e120*omegaR*vx^3*wn*sign(vx)*(vx^2 + vz^2)^(1/2) + 2.27e121*omegaL*vz^3*wn*sign(vx)*(vx^2 + vz^2)^(1/2) + 2.27e121*omegaR*vz^3*wn*sign(vx)*(vx^2 + vz^2)^(1/2) + 2.29e120*omegaL*vx^2*atan2(1.0*vz, vx)*sign(omegaL)*sign(vx) - 2.29e120*omegaR*vx^2*atan2(1.0*vz, vx)*sign(omegaR)*sign(vx) + 2.29e120*omegaL*vy^2*atan2(1.0*vz, vx)*sign(omegaL)*sign(vx) - 2.29e120*omegaR*vy^2*atan2(1.0*vz, vx)*sign(omegaR)*sign(vx) + 2.29e120*omegaL*vz^2*atan2(1.0*vz, vx)*sign(omegaL)*sign(vx) - 2.29e120*omegaR*vz^2*atan2(1.0*vz, vx)*sign(omegaR)*sign(vx) + 1.13e121*deltaL*omegaL*vx^4*wn*sign(vx)^2 + 1.31e118*deltaL*omegaR^3*vx^2*wn*sign(vx) + 1.31e118*deltaR*omegaL^3*vx^2*wn*sign(vx) + 1.13e121*deltaL*omegaR*vx^4*wn*sign(vx)^2 + 1.13e121*deltaR*omegaL*vx^4*wn*sign(vx)^2 + 1.13e121*deltaR*omegaR*vx^4*wn*sign(vx)^2 + 1.13e121*deltaL*omegaL*vy^4*wn*sign(vx)^2 + 1.31e118*deltaL*omegaR^3*vy^2*wn*sign(vx) + 1.31e118*deltaR*omegaL^3*vy^2*wn*sign(vx) + 1.13e121*deltaL*omegaR*vy^4*wn*sign(vx)^2 + 1.13e121*deltaR*omegaL*vy^4*wn*sign(vx)^2 + 1.13e121*deltaR*omegaR*vy^4*wn*sign(vx)^2 + 1.13e121*deltaL*omegaL*vz^4*wn*sign(vx)^2 + 1.31e118*deltaL*omegaR^3*vz^2*wn*sign(vx) + 1.31e118*deltaR*omegaL^3*vz^2*wn*sign(vx) + 1.13e121*deltaL*omegaR*vz^4*wn*sign(vx)^2 + 1.13e121*deltaR*omegaL*vz^4*wn*sign(vx)^2 + 1.13e121*deltaR*omegaR*vz^4*wn*sign(vx)^2 - 1.32e117*omegaL*omegaR^2*wn^2*wz*sign(omegaL) + 1.32e117*omegaL^2*omegaR*wn^2*wz*sign(omegaR) - 1.32e117*omegaL*omegaR^2*wn^2*wzr*sign(omegaL) + 1.32e117*omegaL^2*omegaR*wn^2*wzr*sign(omegaR) - 5.26e119*vy^3*wn*abs(omegaL)*sign(vx)*(vx^2 + vy^2)^(1/2) + 5.26e119*vy^3*wn*abs(omegaR)*sign(vx)*(vx^2 + vy^2)^(1/2) + 3.18e117*omegaL^3*vx*wn*cos(2.0*atan2(1.0*vy, vx))*(vx^2 + vy^2)^(1/2) + 3.18e117*omegaR^3*vx*wn*cos(2.0*atan2(1.0*vy, vx))*(vx^2 + vy^2)^(1/2) + 1.89e117*omegaL^3*vy*wn*cos(2.0*atan2(1.0*vy, vx))*(vx^2 + vy^2)^(1/2) - 1.89e117*omegaR^3*vy*wn*cos(2.0*atan2(1.0*vy, vx))*(vx^2 + vy^2)^(1/2) - 1.28e118*omegaL^3*vz*wn*cos(2.0*atan2(1.0*vz, vx))*(vx^2 + vz^2)^(1/2) - 1.28e118*omegaR^3*vz*wn*cos(2.0*atan2(1.0*vz, vx))*(vx^2 + vz^2)^(1/2) - 2.14e121*omegaL*vx^2*wn^2*wy*sign(vx) - 2.14e121*omegaR*vx^2*wn^2*wy*sign(vx) - 2.14e121*omegaL*vx^2*wn^2*wyr*sign(vx) - 2.14e121*omegaR*vx^2*wn^2*wyr*sign(vx) - 2.14e121*omegaL*vy^2*wn^2*wy*sign(vx) - 2.14e121*omegaR*vy^2*wn^2*wy*sign(vx) - 2.14e121*omegaL*vy^2*wn^2*wyr*sign(vx) - 2.14e121*omegaR*vy^2*wn^2*wyr*sign(vx) - 2.14e121*omegaL*vz^2*wn^2*wy*sign(vx) - 2.14e121*omegaR*vz^2*wn^2*wy*sign(vx) - 2.14e121*omegaL*vz^2*wn^2*wyr*sign(vx) - 2.14e121*omegaR*vz^2*wn^2*wyr*sign(vx) - 1.13e117*omegaL^3*vx*wn*sin(2.0*atan2(1.0*vy, vx))*(vx^2 + vy^2)^(1/2) + 1.13e117*omegaR^3*vx*wn*sin(2.0*atan2(1.0*vy, vx))*(vx^2 + vy^2)^(1/2) + 1.91e117*omegaL^3*vy*wn*sin(2.0*atan2(1.0*vy, vx))*(vx^2 + vy^2)^(1/2) + 1.91e117*omegaR^3*vy*wn*sin(2.0*atan2(1.0*vy, vx))*(vx^2 + vy^2)^(1/2) + 7.66e117*omegaL^3*vx*wn*sin(2.0*atan2(1.0*vz, vx))*(vx^2 + vz^2)^(1/2) + 7.66e117*omegaR^3*vx*wn*sin(2.0*atan2(1.0*vz, vx))*(vx^2 + vz^2)^(1/2) - 1.85e120*a11*omegaL*omegaR^2*wn*wx + 1.85e120*a11*omegaL^2*omegaR*wn*wx - 1.85e120*b11*omegaL*omegaR^2*wn*wz + 1.85e120*b11*omegaL^2*omegaR*wn*wz + 1.85e120*a21*omegaL^3*vx*wn*wx - 1.85e120*a21*omegaR^3*vx*wn*wx + 1.85e120*a12*omegaL^3*vz*wn*wx - 1.85e120*a12*omegaR^3*vz*wn*wx + 1.85e120*b21*omegaL^3*vx*wn*wz - 1.85e120*b21*omegaR^3*vx*wn*wz + 1.85e120*b12*omegaL^3*vz*wn*wz - 1.85e120*b12*omegaR^3*vz*wn*wz - 3.18e117*omegaL*omegaR^2*vx*wn*(vx^2 + vy^2)^(1/2) - 3.18e117*omegaL^2*omegaR*vx*wn*(vx^2 + vy^2)^(1/2) + 1.28e117*omegaL*omegaR^2*vx*wn*(vx^2 + vz^2)^(1/2) + 1.89e117*omegaL*omegaR^2*vy*wn*(vx^2 + vy^2)^(1/2) + 1.28e117*omegaL^2*omegaR*vx*wn*(vx^2 + vz^2)^(1/2) - 1.89e117*omegaL^2*omegaR*vy*wn*(vx^2 + vy^2)^(1/2) + 1.31e118*omegaL*omegaR^2*vz*wn*(vx^2 + vz^2)^(1/2) + 1.31e118*omegaL^2*omegaR*vz*wn*(vx^2 + vz^2)^(1/2) + 6.38e119*omegaL*omegaR^2*wn*wy*(vx^2 + vz^2)^(1/2) + 6.38e119*omegaL^2*omegaR*wn*wy*(vx^2 + vz^2)^(1/2) + 5.26e119*vy^3*wn*cos(2.0*atan2(1.0*vy, vx))*abs(omegaL)*sign(vx)*(vx^2 + vy^2)^(1/2) - 5.26e119*vy^3*wn*cos(2.0*atan2(1.0*vy, vx))*abs(omegaR)*sign(vx)*(vx^2 + vy^2)^(1/2) - 3.3e118*c31*omegaL^2*vx^2*wn*wz*abs(omegaL) + 3.3e118*c31*omegaL^2*vx^2*wn*wz*abs(omegaR) - 3.3e118*c31*omegaR^2*vx^2*wn*wz*abs(omegaL) - 3.3e118*c41*omegaL^2*vx^3*wn*wz*abs(omegaL) + 3.3e118*c31*omegaR^2*vx^2*wn*wz*abs(omegaR) + 3.3e118*c41*omegaL^2*vx^3*wn*wz*abs(omegaR) - 3.3e118*c41*omegaR^2*vx^3*wn*wz*abs(omegaL) + 3.3e118*c41*omegaR^2*vx^3*wn*wz*abs(omegaR) - 3.3e118*c13*omegaL^2*vz^2*wn*wz*abs(omegaL) - 3.3e118*c14*omegaL^2*vz^3*wn*wz*abs(omegaL) + 3.3e118*c13*omegaL^2*vz^2*wn*wz*abs(omegaR) - 3.3e118*c13*omegaR^2*vz^2*wn*wz*abs(omegaL) + 3.3e118*c14*omegaL^2*vz^3*wn*wz*abs(omegaR) - 3.3e118*c14*omegaR^2*vz^3*wn*wz*abs(omegaL) + 3.3e118*c13*omegaR^2*vz^2*wn*wz*abs(omegaR) + 3.3e118*c14*omegaR^2*vz^3*wn*wz*abs(omegaR) + 1.85e120*a33*omegaL^3*vx^2*vz^2*wn*wx - 1.85e120*a33*omegaR^3*vx^2*vz^2*wn*wx + 1.85e120*a43*omegaL^3*vx^3*vz^2*wn*wx - 1.85e120*a43*omegaR^3*vx^3*vz^2*wn*wx + 1.85e120*b33*omegaL^3*vx^2*vz^2*wn*wz + 1.85e120*b34*omegaL^3*vx^2*vz^3*wn*wz - 1.85e120*b33*omegaR^3*vx^2*vz^2*wn*wz - 1.85e120*b34*omegaR^3*vx^2*vz^3*wn*wz - 3.16e119*vx^3*wn*sin(2.0*atan2(1.0*vy, vx))*abs(omegaL)*sign(vx)*(vx^2 + vy^2)^(1/2) + 3.16e119*vx^3*wn*sin(2.0*atan2(1.0*vy, vx))*abs(omegaR)*sign(vx)*(vx^2 + vy^2)^(1/2) - 3.3e118*c31*omegaL^3*vx^2*wn*wz*sign(omegaL) - 3.3e118*c41*omegaL^3*vx^3*wn*wz*sign(omegaL) + 3.3e118*c31*omegaR^3*vx^2*wn*wz*sign(omegaR) + 3.3e118*c41*omegaR^3*vx^3*wn*wz*sign(omegaR) - 3.3e118*c13*omegaL^3*vz^2*wn*wz*sign(omegaL) - 3.3e118*c14*omegaL^3*vz^3*wn*wz*sign(omegaL) + 3.3e118*c13*omegaR^3*vz^2*wn*wz*sign(omegaR) + 3.3e118*c14*omegaR^3*vz^3*wn*wz*sign(omegaR) + 2.61e118*deltaL*omegaL*omegaR^2*vx^2*wn*sign(vx) + 1.31e118*deltaL*omegaL^2*omegaR*vx^2*wn*sign(vx) + 1.31e118*deltaR*omegaL*omegaR^2*vx^2*wn*sign(vx) + 2.61e118*deltaR*omegaL^2*omegaR*vx^2*wn*sign(vx) + 2.61e118*deltaL*omegaL*omegaR^2*vy^2*wn*sign(vx) + 1.31e118*deltaL*omegaL^2*omegaR*vy^2*wn*sign(vx) + 1.31e118*deltaR*omegaL*omegaR^2*vy^2*wn*sign(vx) + 2.61e118*deltaR*omegaL^2*omegaR*vy^2*wn*sign(vx) + 2.61e118*deltaL*omegaL*omegaR^2*vz^2*wn*sign(vx) + 1.31e118*deltaL*omegaL^2*omegaR*vz^2*wn*sign(vx) + 1.31e118*deltaR*omegaL*omegaR^2*vz^2*wn*sign(vx) + 2.61e118*deltaR*omegaL^2*omegaR*vz^2*wn*sign(vx) - 5.19e121*deltaL*omegaL*vx^2*wn^2*wz*sign(vx) + 5.19e121*deltaR*omegaR*vx^2*wn^2*wz*sign(vx) - 5.19e121*deltaL*omegaL*vx^2*wn^2*wzr*sign(vx) + 5.19e121*deltaR*omegaR*vx^2*wn^2*wzr*sign(vx) - 5.19e121*deltaL*omegaL*vy^2*wn^2*wz*sign(vx) + 5.19e121*deltaR*omegaR*vy^2*wn^2*wz*sign(vx) - 5.19e121*deltaL*omegaL*vy^2*wn^2*wzr*sign(vx) + 5.19e121*deltaR*omegaR*vy^2*wn^2*wzr*sign(vx) - 5.19e121*deltaL*omegaL*vz^2*wn^2*wz*sign(vx) + 5.19e121*deltaR*omegaR*vz^2*wn^2*wz*sign(vx) - 5.19e121*deltaL*omegaL*vz^2*wn^2*wzr*sign(vx) + 5.19e121*deltaR*omegaR*vz^2*wn^2*wzr*sign(vx) - 5.74e121*c11*vx^2*wn*wz*abs(omegaL)*sign(vx) + 5.74e121*c11*vx^2*wn*wz*abs(omegaR)*sign(vx) - 5.74e121*c21*vx^3*wn*wz*abs(omegaL)*sign(vx) + 5.74e121*c21*vx^3*wn*wz*abs(omegaR)*sign(vx) - 5.74e121*c31*vx^4*wn*wz*abs(omegaL)*sign(vx) + 5.74e121*c31*vx^4*wn*wz*abs(omegaR)*sign(vx) - 5.74e121*c41*vx^5*wn*wz*abs(omegaL)*sign(vx) + 5.74e121*c41*vx^5*wn*wz*abs(omegaR)*sign(vx) - 5.74e121*c11*vy^2*wn*wz*abs(omegaL)*sign(vx) + 5.74e121*c11*vy^2*wn*wz*abs(omegaR)*sign(vx) - 5.74e121*c11*vz^2*wn*wz*abs(omegaL)*sign(vx) - 5.74e121*c12*vz^3*wn*wz*abs(omegaL)*sign(vx) - 5.74e121*c13*vz^4*wn*wz*abs(omegaL)*sign(vx) + 5.74e121*c11*vz^2*wn*wz*abs(omegaR)*sign(vx) - 5.74e121*c14*vz^5*wn*wz*abs(omegaL)*sign(vx) + 5.74e121*c12*vz^3*wn*wz*abs(omegaR)*sign(vx) + 5.74e121*c13*vz^4*wn*wz*abs(omegaR)*sign(vx) + 5.74e121*c14*vz^5*wn*wz*abs(omegaR)*sign(vx) + 1.15e117*omegaL*omegaR*vx^2*wn*abs(omegaL)*sign(vx) + 1.15e117*omegaL*omegaR*vx^2*wn*abs(omegaR)*sign(vx) + 1.15e117*omegaL*omegaR*vy^2*wn*abs(omegaL)*sign(vx) + 1.15e117*omegaL*omegaR*vy^2*wn*abs(omegaR)*sign(vx) + 1.15e117*omegaL*omegaR*vz^2*wn*abs(omegaL)*sign(vx) + 1.15e117*omegaL*omegaR*vz^2*wn*abs(omegaR)*sign(vx) + 3.18e117*omegaL*omegaR^2*vx*wn*cos(2.0*atan2(1.0*vy, vx))*(vx^2 + vy^2)^(1/2) + 3.18e117*omegaL^2*omegaR*vx*wn*cos(2.0*atan2(1.0*vy, vx))*(vx^2 + vy^2)^(1/2) - 1.89e117*omegaL*omegaR^2*vy*wn*cos(2.0*atan2(1.0*vy, vx))*(vx^2 + vy^2)^(1/2) + 1.89e117*omegaL^2*omegaR*vy*wn*cos(2.0*atan2(1.0*vy, vx))*(vx^2 + vy^2)^(1/2) - 1.28e118*omegaL*omegaR^2*vz*wn*cos(2.0*atan2(1.0*vz, vx))*(vx^2 + vz^2)^(1/2) - 1.28e118*omegaL^2*omegaR*vz*wn*cos(2.0*atan2(1.0*vz, vx))*(vx^2 + vz^2)^(1/2) - 5.26e119*vx^2*vy*wn*abs(omegaL)*sign(vx)*(vx^2 + vy^2)^(1/2) + 5.26e119*vx^2*vy*wn*abs(omegaR)*sign(vx)*(vx^2 + vy^2)^(1/2) - 5.26e119*vy*vz^2*wn*abs(omegaL)*sign(vx)*(vx^2 + vy^2)^(1/2) + 5.26e119*vy*vz^2*wn*abs(omegaR)*sign(vx)*(vx^2 + vy^2)^(1/2) - 5.26e119*omegaL*vy^3*wn*sign(omegaL)*sign(vx)*(vx^2 + vy^2)^(1/2) + 5.26e119*omegaR*vy^3*wn*sign(omegaR)*sign(vx)*(vx^2 + vy^2)^(1/2) - 1.49e120*c11*deltaL*omegaL*omegaR^2*wn*wz + 1.49e120*c11*deltaR*omegaL^2*omegaR*wn*wz + 1.13e117*omegaL*omegaR^2*vx*wn*sin(2.0*atan2(1.0*vy, vx))*(vx^2 + vy^2)^(1/2) - 1.13e117*omegaL^2*omegaR*vx*wn*sin(2.0*atan2(1.0*vy, vx))*(vx^2 + vy^2)^(1/2) + 1.91e117*omegaL*omegaR^2*vy*wn*sin(2.0*atan2(1.0*vy, vx))*(vx^2 + vy^2)^(1/2) + 1.91e117*omegaL^2*omegaR*vy*wn*sin(2.0*atan2(1.0*vy, vx))*(vx^2 + vy^2)^(1/2) + 7.66e117*omegaL*omegaR^2*vx*wn*sin(2.0*atan2(1.0*vz, vx))*(vx^2 + vz^2)^(1/2) + 7.66e117*omegaL^2*omegaR*vx*wn*sin(2.0*atan2(1.0*vz, vx))*(vx^2 + vz^2)^(1/2) - 1.37e118*deltaL*omegaL*omegaR^2*vy*wn*(vx^2 + vy^2)^(1/2) + 1.37e118*deltaR*omegaL^2*omegaR*vy*wn*(vx^2 + vy^2)^(1/2) - 1.85e120*a21*omegaL*omegaR^2*vx*wn*wx + 1.85e120*a21*omegaL^2*omegaR*vx*wn*wx - 1.85e120*a12*omegaL*omegaR^2*vz*wn*wx + 1.85e120*a12*omegaL^2*omegaR*vz*wn*wx - 1.85e120*b21*omegaL*omegaR^2*vx*wn*wz + 1.85e120*b21*omegaL^2*omegaR*vx*wn*wz - 1.85e120*b12*omegaL*omegaR^2*vz*wn*wz + 1.85e120*b12*omegaL^2*omegaR*vz*wn*wz + 1.85e120*a22*omegaL^3*vx*vz*wn*wx - 1.85e120*a22*omegaR^3*vx*vz*wn*wx + 1.85e120*b22*omegaL^3*vx*vz*wn*wz - 1.85e120*b22*omegaR^3*vx*vz*wn*wz + 2.27e121*deltaL*omegaL*vx^2*vy^2*wn*sign(vx)^2 + 2.27e121*deltaL*omegaR*vx^2*vy^2*wn*sign(vx)^2 + 2.27e121*deltaR*omegaL*vx^2*vy^2*wn*sign(vx)^2 + 2.27e121*deltaR*omegaR*vx^2*vy^2*wn*sign(vx)^2 + 2.27e121*deltaL*omegaL*vx^2*vz^2*wn*sign(vx)^2 + 2.27e121*deltaL*omegaR*vx^2*vz^2*wn*sign(vx)^2 + 2.27e121*deltaR*omegaL*vx^2*vz^2*wn*sign(vx)^2 + 2.27e121*deltaR*omegaR*vx^2*vz^2*wn*sign(vx)^2 + 2.27e121*deltaL*omegaL*vy^2*vz^2*wn*sign(vx)^2 + 2.27e121*deltaL*omegaR*vy^2*vz^2*wn*sign(vx)^2 + 2.27e121*deltaR*omegaL*vy^2*vz^2*wn*sign(vx)^2 + 2.27e121*deltaR*omegaR*vy^2*vz^2*wn*sign(vx)^2 + 3.03e116*omegaL^2*vy*wn*cos(2.0*atan2(1.0*vy, vx))*abs(omegaL)*(vx^2 + vy^2)^(1/2) - 3.03e116*omegaL^2*vy*wn*cos(2.0*atan2(1.0*vy, vx))*abs(omegaR)*(vx^2 + vy^2)^(1/2) + 3.03e116*omegaR^2*vy*wn*cos(2.0*atan2(1.0*vy, vx))*abs(omegaL)*(vx^2 + vy^2)^(1/2) - 3.03e116*omegaR^2*vy*wn*cos(2.0*atan2(1.0*vy, vx))*abs(omegaR)*(vx^2 + vy^2)^(1/2) + 5.77e116*omegaL*omegaR^2*vx^2*wn*sign(omegaL)*sign(vx) + 5.77e116*omegaL^2*omegaR*vx^2*wn*sign(omegaR)*sign(vx) + 5.77e116*omegaL*omegaR^2*vy^2*wn*sign(omegaL)*sign(vx) + 5.77e116*omegaL^2*omegaR*vy^2*wn*sign(omegaR)*sign(vx) + 5.77e116*omegaL*omegaR^2*vz^2*wn*sign(omegaL)*sign(vx) + 5.77e116*omegaL^2*omegaR*vz^2*wn*sign(omegaR)*sign(vx) - 1.82e116*omegaL^2*vx*wn*sin(2.0*atan2(1.0*vy, vx))*abs(omegaL)*(vx^2 + vy^2)^(1/2) + 1.82e116*omegaL^2*vx*wn*sin(2.0*atan2(1.0*vy, vx))*abs(omegaR)*(vx^2 + vy^2)^(1/2) - 1.82e116*omegaR^2*vx*wn*sin(2.0*atan2(1.0*vy, vx))*abs(omegaL)*(vx^2 + vy^2)^(1/2) + 1.82e116*omegaR^2*vx*wn*sin(2.0*atan2(1.0*vy, vx))*abs(omegaR)*(vx^2 + vy^2)^(1/2) + 3.03e116*omegaL^3*vy*wn*cos(2.0*atan2(1.0*vy, vx))*sign(omegaL)*(vx^2 + vy^2)^(1/2) - 3.03e116*omegaR^3*vy*wn*cos(2.0*atan2(1.0*vy, vx))*sign(omegaR)*(vx^2 + vy^2)^(1/2) - 2.29e120*omegaL*vx^2*wn^2*wz*sign(omegaL)*sign(vx) + 2.29e120*omegaR*vx^2*wn^2*wz*sign(omegaR)*sign(vx) - 2.29e120*omegaL*vx^2*wn^2*wzr*sign(omegaL)*sign(vx) + 2.29e120*omegaR*vx^2*wn^2*wzr*sign(omegaR)*sign(vx) - 2.29e120*omegaL*vy^2*wn^2*wz*sign(omegaL)*sign(vx) + 2.29e120*omegaR*vy^2*wn^2*wz*sign(omegaR)*sign(vx) - 2.29e120*omegaL*vy^2*wn^2*wzr*sign(omegaL)*sign(vx) + 2.29e120*omegaR*vy^2*wn^2*wzr*sign(omegaR)*sign(vx) - 2.29e120*omegaL*vz^2*wn^2*wz*sign(omegaL)*sign(vx) + 2.29e120*omegaR*vz^2*wn^2*wz*sign(omegaR)*sign(vx) - 2.29e120*omegaL*vz^2*wn^2*wzr*sign(omegaL)*sign(vx) + 2.29e120*omegaR*vz^2*wn^2*wzr*sign(omegaR)*sign(vx) + 5.52e120*omegaL*vx^3*wn*cos(2.0*atan2(1.0*vy, vx))*sign(vx)*(vx^2 + vy^2)^(1/2) + 5.52e120*omegaR*vx^3*wn*cos(2.0*atan2(1.0*vy, vx))*sign(vx)*(vx^2 + vy^2)^(1/2) - 2.22e121*omegaL*vz^3*wn*cos(2.0*atan2(1.0*vz, vx))*sign(vx)*(vx^2 + vz^2)^(1/2) - 2.22e121*omegaR*vz^3*wn*cos(2.0*atan2(1.0*vz, vx))*sign(vx)*(vx^2 + vz^2)^(1/2) - 1.85e120*a31*omegaL*omegaR^2*vx^2*wn*wx + 1.85e120*a31*omegaL^2*omegaR*vx^2*wn*wx - 1.85e120*a41*omegaL*omegaR^2*vx^3*wn*wx + 1.85e120*a41*omegaL^2*omegaR*vx^3*wn*wx - 1.85e120*a13*omegaL*omegaR^2*vz^2*wn*wx + 1.85e120*a13*omegaL^2*omegaR*vz^2*wn*wx - 1.85e120*b31*omegaL*omegaR^2*vx^2*wn*wz + 1.85e120*b31*omegaL^2*omegaR*vx^2*wn*wz - 1.85e120*b13*omegaL*omegaR^2*vz^2*wn*wz + 1.85e120*b13*omegaL^2*omegaR*vz^2*wn*wz - 1.85e120*b14*omegaL*omegaR^2*vz^3*wn*wz + 1.85e120*b14*omegaL^2*omegaR*vz^3*wn*wz - 3.3e118*c21*omegaL^2*vx*wn*wz*abs(omegaL) + 3.3e118*c21*omegaL^2*vx*wn*wz*abs(omegaR) - 3.3e118*c21*omegaR^2*vx*wn*wz*abs(omegaL) + 3.3e118*c21*omegaR^2*vx*wn*wz*abs(omegaR) - 3.3e118*c12*omegaL^2*vz*wn*wz*abs(omegaL) + 3.3e118*c12*omegaL^2*vz*wn*wz*abs(omegaR) - 3.3e118*c12*omegaR^2*vz*wn*wz*abs(omegaL) + 3.3e118*c12*omegaR^2*vz*wn*wz*abs(omegaR) - 1.82e116*omegaL^3*vx*wn*sin(2.0*atan2(1.0*vy, vx))*sign(omegaL)*(vx^2 + vy^2)^(1/2) + 1.82e116*omegaR^3*vx*wn*sin(2.0*atan2(1.0*vy, vx))*sign(omegaR)*(vx^2 + vy^2)^(1/2) + 1.85e120*a23*omegaL^3*vx*vz^2*wn*wx - 1.85e120*a23*omegaR^3*vx*vz^2*wn*wx + 1.85e120*a32*omegaL^3*vx^2*vz*wn*wx - 1.85e120*a32*omegaR^3*vx^2*vz*wn*wx + 1.85e120*a42*omegaL^3*vx^3*vz*wn*wx - 1.85e120*a42*omegaR^3*vx^3*vz*wn*wx + 1.85e120*b23*omegaL^3*vx*vz^2*wn*wz + 1.85e120*b24*omegaL^3*vx*vz^3*wn*wz - 1.85e120*b23*omegaR^3*vx*vz^2*wn*wz - 1.85e120*b24*omegaR^3*vx*vz^3*wn*wz + 1.85e120*b32*omegaL^3*vx^2*vz*wn*wz - 1.85e120*b32*omegaR^3*vx^2*vz*wn*wz + 3.31e120*omegaL*vy^3*wn*sin(2.0*atan2(1.0*vy, vx))*sign(vx)*(vx^2 + vy^2)^(1/2) + 3.31e120*omegaR*vy^3*wn*sin(2.0*atan2(1.0*vy, vx))*sign(vx)*(vx^2 + vy^2)^(1/2) + 1.33e121*omegaL*vx^3*wn*sin(2.0*atan2(1.0*vz, vx))*sign(vx)*(vx^2 + vz^2)^(1/2) + 1.33e121*omegaR*vx^3*wn*sin(2.0*atan2(1.0*vz, vx))*sign(vx)*(vx^2 + vz^2)^(1/2) - 3.3e118*c11*omegaL*omegaR^2*wn*wz*sign(omegaL) + 3.3e118*c11*omegaL^2*omegaR*wn*wz*sign(omegaR) - 1.19e121*deltaL*omegaL*vy^3*wn*sign(vx)*(vx^2 + vy^2)^(1/2) + 1.19e121*deltaR*omegaR*vy^3*wn*sign(vx)*(vx^2 + vy^2)^(1/2) - 3.03e116*omegaL*omegaR^2*vy*wn*sign(omegaL)*(vx^2 + vy^2)^(1/2) + 3.03e116*omegaL^2*omegaR*vy*wn*sign(omegaR)*(vx^2 + vy^2)^(1/2) - 3.3e118*c21*omegaL^3*vx*wn*wz*sign(omegaL) + 3.3e118*c21*omegaR^3*vx*wn*wz*sign(omegaR) - 3.3e118*c12*omegaL^3*vz*wn*wz*sign(omegaL) + 3.3e118*c12*omegaR^3*vz*wn*wz*sign(omegaR) - 5.52e120*omegaL*vx*vy^2*wn*sign(vx)*(vx^2 + vy^2)^(1/2) - 5.52e120*omegaR*vx*vy^2*wn*sign(vx)*(vx^2 + vy^2)^(1/2) + 2.22e120*omegaL*vx*vy^2*wn*sign(vx)*(vx^2 + vz^2)^(1/2) - 5.52e120*omegaL*vx*vz^2*wn*sign(vx)*(vx^2 + vy^2)^(1/2) + 2.22e120*omegaR*vx*vy^2*wn*sign(vx)*(vx^2 + vz^2)^(1/2) - 5.52e120*omegaR*vx*vz^2*wn*sign(vx)*(vx^2 + vy^2)^(1/2) + 2.22e120*omegaL*vx*vz^2*wn*sign(vx)*(vx^2 + vz^2)^(1/2) + 2.27e121*omegaL*vx^2*vz*wn*sign(vx)*(vx^2 + vz^2)^(1/2) + 2.22e120*omegaR*vx*vz^2*wn*sign(vx)*(vx^2 + vz^2)^(1/2) + 2.27e121*omegaR*vx^2*vz*wn*sign(vx)*(vx^2 + vz^2)^(1/2) + 2.27e121*omegaL*vy^2*vz*wn*sign(vx)*(vx^2 + vz^2)^(1/2) + 2.27e121*omegaR*vy^2*vz*wn*sign(vx)*(vx^2 + vz^2)^(1/2) + 1.11e123*omegaL*vx^2*wn*wy*sign(vx)*(vx^2 + vz^2)^(1/2) + 1.11e123*omegaR*vx^2*wn*wy*sign(vx)*(vx^2 + vz^2)^(1/2) + 1.11e123*omegaL*vy^2*wn*wy*sign(vx)*(vx^2 + vz^2)^(1/2) + 1.11e123*omegaR*vy^2*wn*wy*sign(vx)*(vx^2 + vz^2)^(1/2) + 1.11e123*omegaL*vz^2*wn*wy*sign(vx)*(vx^2 + vz^2)^(1/2) + 1.11e123*omegaR*vz^2*wn*wy*sign(vx)*(vx^2 + vz^2)^(1/2) - 3.3e118*c33*omegaL^3*vx^2*vz^2*wn*wz*sign(omegaL) - 3.3e118*c34*omegaL^3*vx^2*vz^3*wn*wz*sign(omegaL) - 3.3e118*c43*omegaL^3*vx^3*vz^2*wn*wz*sign(omegaL) + 3.3e118*c33*omegaR^3*vx^2*vz^2*wn*wz*sign(omegaR) - 3.3e118*c44*omegaL^3*vx^3*vz^3*wn*wz*sign(omegaL) + 3.3e118*c34*omegaR^3*vx^2*vz^3*wn*wz*sign(omegaR) + 3.3e118*c43*omegaR^3*vx^3*vz^2*wn*wz*sign(omegaR) + 3.3e118*c44*omegaR^3*vx^3*vz^3*wn*wz*sign(omegaR) - 5.74e121*c31*vx^2*vy^2*wn*wz*abs(omegaL)*sign(vx) + 5.74e121*c31*vx^2*vy^2*wn*wz*abs(omegaR)*sign(vx) - 5.74e121*c41*vx^3*vy^2*wn*wz*abs(omegaL)*sign(vx) + 5.74e121*c41*vx^3*vy^2*wn*wz*abs(omegaR)*sign(vx) - 5.74e121*c13*vx^2*vz^2*wn*wz*abs(omegaL)*sign(vx) - 5.74e121*c14*vx^2*vz^3*wn*wz*abs(omegaL)*sign(vx) + 5.74e121*c13*vx^2*vz^2*wn*wz*abs(omegaR)*sign(vx) + 5.74e121*c14*vx^2*vz^3*wn*wz*abs(omegaR)*sign(vx) - 5.74e121*c23*vx^3*vz^2*wn*wz*abs(omegaL)*sign(vx) - 5.74e121*c24*vx^3*vz^3*wn*wz*abs(omegaL)*sign(vx) + 5.74e121*c23*vx^3*vz^2*wn*wz*abs(omegaR)*sign(vx) - 5.74e121*c31*vx^2*vz^2*wn*wz*abs(omegaL)*sign(vx) + 5.74e121*c24*vx^3*vz^3*wn*wz*abs(omegaR)*sign(vx) - 5.74e121*c32*vx^2*vz^3*wn*wz*abs(omegaL)*sign(vx) - 5.74e121*c33*vx^2*vz^4*wn*wz*abs(omegaL)*sign(vx) - 5.74e121*c33*vx^4*vz^2*wn*wz*abs(omegaL)*sign(vx) + 5.74e121*c31*vx^2*vz^2*wn*wz*abs(omegaR)*sign(vx) - 5.74e121*c34*vx^2*vz^5*wn*wz*abs(omegaL)*sign(vx) - 5.74e121*c34*vx^4*vz^3*wn*wz*abs(omegaL)*sign(vx) + 5.74e121*c32*vx^2*vz^3*wn*wz*abs(omegaR)*sign(vx) + 5.74e121*c33*vx^2*vz^4*wn*wz*abs(omegaR)*sign(vx) + 5.74e121*c33*vx^4*vz^2*wn*wz*abs(omegaR)*sign(vx) - 5.74e121*c41*vx^3*vz^2*wn*wz*abs(omegaL)*sign(vx) + 5.74e121*c34*vx^2*vz^5*wn*wz*abs(omegaR)*sign(vx) + 5.74e121*c34*vx^4*vz^3*wn*wz*abs(omegaR)*sign(vx) - 5.74e121*c42*vx^3*vz^3*wn*wz*abs(omegaL)*sign(vx) - 5.74e121*c43*vx^3*vz^4*wn*wz*abs(omegaL)*sign(vx) - 5.74e121*c43*vx^5*vz^2*wn*wz*abs(omegaL)*sign(vx) + 5.74e121*c41*vx^3*vz^2*wn*wz*abs(omegaR)*sign(vx) - 5.74e121*c44*vx^3*vz^5*wn*wz*abs(omegaL)*sign(vx) - 5.74e121*c44*vx^5*vz^3*wn*wz*abs(omegaL)*sign(vx) + 5.74e121*c42*vx^3*vz^3*wn*wz*abs(omegaR)*sign(vx) + 5.74e121*c43*vx^3*vz^4*wn*wz*abs(omegaR)*sign(vx) + 5.74e121*c43*vx^5*vz^2*wn*wz*abs(omegaR)*sign(vx) + 5.74e121*c44*vx^3*vz^5*wn*wz*abs(omegaR)*sign(vx) + 5.74e121*c44*vx^5*vz^3*wn*wz*abs(omegaR)*sign(vx) - 5.74e121*c13*vy^2*vz^2*wn*wz*abs(omegaL)*sign(vx) - 5.74e121*c14*vy^2*vz^3*wn*wz*abs(omegaL)*sign(vx) + 5.74e121*c13*vy^2*vz^2*wn*wz*abs(omegaR)*sign(vx) + 5.74e121*c14*vy^2*vz^3*wn*wz*abs(omegaR)*sign(vx) + 1.19e121*deltaL*omegaL*vy^3*wn*cos(2.0*atan2(1.0*vy, vx))*sign(vx)*(vx^2 + vy^2)^(1/2) - 1.19e121*deltaR*omegaR*vy^3*wn*cos(2.0*atan2(1.0*vy, vx))*sign(vx)*(vx^2 + vy^2)^(1/2) + 3.03e116*omegaL*omegaR^2*vy*wn*cos(2.0*atan2(1.0*vy, vx))*sign(omegaL)*(vx^2 + vy^2)^(1/2) - 3.03e116*omegaL^2*omegaR*vy*wn*cos(2.0*atan2(1.0*vy, vx))*sign(omegaR)*(vx^2 + vy^2)^(1/2) - 1.49e120*c31*deltaL*omegaL*omegaR^2*vx^2*wn*wz + 1.49e120*c31*deltaR*omegaL^2*omegaR*vx^2*wn*wz - 1.49e120*c41*deltaL*omegaL*omegaR^2*vx^3*wn*wz + 1.49e120*c41*deltaR*omegaL^2*omegaR*vx^3*wn*wz - 1.49e120*c13*deltaL*omegaL*omegaR^2*vz^2*wn*wz - 1.49e120*c14*deltaL*omegaL*omegaR^2*vz^3*wn*wz + 1.49e120*c13*deltaR*omegaL^2*omegaR*vz^2*wn*wz + 1.49e120*c14*deltaR*omegaL^2*omegaR*vz^3*wn*wz - 7.14e120*deltaL*omegaL*vx^3*wn*sin(2.0*atan2(1.0*vy, vx))*sign(vx)*(vx^2 + vy^2)^(1/2) + 7.14e120*deltaR*omegaR*vx^3*wn*sin(2.0*atan2(1.0*vy, vx))*sign(vx)*(vx^2 + vy^2)^(1/2) + 5.52e120*omegaL*vx*vy^2*wn*cos(2.0*atan2(1.0*vy, vx))*sign(vx)*(vx^2 + vy^2)^(1/2) + 5.52e120*omegaR*vx*vy^2*wn*cos(2.0*atan2(1.0*vy, vx))*sign(vx)*(vx^2 + vy^2)^(1/2) + 5.52e120*omegaL*vx*vz^2*wn*cos(2.0*atan2(1.0*vy, vx))*sign(vx)*(vx^2 + vy^2)^(1/2) + 5.52e120*omegaR*vx*vz^2*wn*cos(2.0*atan2(1.0*vy, vx))*sign(vx)*(vx^2 + vy^2)^(1/2) - 2.22e121*omegaL*vx^2*vz*wn*cos(2.0*atan2(1.0*vz, vx))*sign(vx)*(vx^2 + vz^2)^(1/2) - 2.22e121*omegaR*vx^2*vz*wn*cos(2.0*atan2(1.0*vz, vx))*sign(vx)*(vx^2 + vz^2)^(1/2) - 2.22e121*omegaL*vy^2*vz*wn*cos(2.0*atan2(1.0*vz, vx))*sign(vx)*(vx^2 + vz^2)^(1/2) - 2.22e121*omegaR*vy^2*vz*wn*cos(2.0*atan2(1.0*vz, vx))*sign(vx)*(vx^2 + vz^2)^(1/2) - 1.82e116*omegaL*omegaR^2*vx*wn*sin(2.0*atan2(1.0*vy, vx))*sign(omegaL)*(vx^2 + vy^2)^(1/2) + 1.82e116*omegaL^2*omegaR*vx*wn*sin(2.0*atan2(1.0*vy, vx))*sign(omegaR)*(vx^2 + vy^2)^(1/2) - 1.85e120*a23*omegaL*omegaR^2*vx*vz^2*wn*wx + 1.85e120*a23*omegaL^2*omegaR*vx*vz^2*wn*wx - 1.85e120*a32*omegaL*omegaR^2*vx^2*vz*wn*wx + 1.85e120*a32*omegaL^2*omegaR*vx^2*vz*wn*wx - 1.85e120*a42*omegaL*omegaR^2*vx^3*vz*wn*wx + 1.85e120*a42*omegaL^2*omegaR*vx^3*vz*wn*wx - 1.85e120*b23*omegaL*omegaR^2*vx*vz^2*wn*wz + 1.85e120*b23*omegaL^2*omegaR*vx*vz^2*wn*wz - 1.85e120*b24*omegaL*omegaR^2*vx*vz^3*wn*wz + 1.85e120*b24*omegaL^2*omegaR*vx*vz^3*wn*wz - 1.85e120*b32*omegaL*omegaR^2*vx^2*vz*wn*wz + 1.85e120*b32*omegaL^2*omegaR*vx^2*vz*wn*wz - 3.3e118*c22*omegaL^2*vx*vz*wn*wz*abs(omegaL) + 3.3e118*c22*omegaL^2*vx*vz*wn*wz*abs(omegaR) - 3.3e118*c22*omegaR^2*vx*vz*wn*wz*abs(omegaL) + 3.3e118*c22*omegaR^2*vx*vz*wn*wz*abs(omegaR) - 1.3e123*c11*deltaL*omegaL*vx^2*wn*wz*sign(vx) - 1.3e123*c21*deltaL*omegaL*vx^3*wn*wz*sign(vx) + 1.3e123*c11*deltaR*omegaR*vx^2*wn*wz*sign(vx) - 1.3e123*c31*deltaL*omegaL*vx^4*wn*wz*sign(vx) + 1.3e123*c21*deltaR*omegaR*vx^3*wn*wz*sign(vx) - 1.3e123*c41*deltaL*omegaL*vx^5*wn*wz*sign(vx) + 1.3e123*c31*deltaR*omegaR*vx^4*wn*wz*sign(vx) + 1.3e123*c41*deltaR*omegaR*vx^5*wn*wz*sign(vx) - 1.3e123*c11*deltaL*omegaL*vy^2*wn*wz*sign(vx) + 1.3e123*c11*deltaR*omegaR*vy^2*wn*wz*sign(vx) - 1.3e123*c11*deltaL*omegaL*vz^2*wn*wz*sign(vx) - 1.3e123*c12*deltaL*omegaL*vz^3*wn*wz*sign(vx) - 1.3e123*c13*deltaL*omegaL*vz^4*wn*wz*sign(vx) - 1.3e123*c14*deltaL*omegaL*vz^5*wn*wz*sign(vx) + 1.3e123*c11*deltaR*omegaR*vz^2*wn*wz*sign(vx) + 1.3e123*c12*deltaR*omegaR*vz^3*wn*wz*sign(vx) + 1.3e123*c13*deltaR*omegaR*vz^4*wn*wz*sign(vx) + 1.3e123*c14*deltaR*omegaR*vz^5*wn*wz*sign(vx) + 3.31e120*omegaL*vx^2*vy*wn*sin(2.0*atan2(1.0*vy, vx))*sign(vx)*(vx^2 + vy^2)^(1/2) + 3.31e120*omegaR*vx^2*vy*wn*sin(2.0*atan2(1.0*vy, vx))*sign(vx)*(vx^2 + vy^2)^(1/2) + 1.33e121*omegaL*vx*vy^2*wn*sin(2.0*atan2(1.0*vz, vx))*sign(vx)*(vx^2 + vz^2)^(1/2) + 3.31e120*omegaL*vy*vz^2*wn*sin(2.0*atan2(1.0*vy, vx))*sign(vx)*(vx^2 + vy^2)^(1/2) + 1.33e121*omegaR*vx*vy^2*wn*sin(2.0*atan2(1.0*vz, vx))*sign(vx)*(vx^2 + vz^2)^(1/2) + 3.31e120*omegaR*vy*vz^2*wn*sin(2.0*atan2(1.0*vy, vx))*sign(vx)*(vx^2 + vy^2)^(1/2) + 1.33e121*omegaL*vx*vz^2*wn*sin(2.0*atan2(1.0*vz, vx))*sign(vx)*(vx^2 + vz^2)^(1/2) + 1.33e121*omegaR*vx*vz^2*wn*sin(2.0*atan2(1.0*vz, vx))*sign(vx)*(vx^2 + vz^2)^(1/2) - 3.3e118*c21*omegaL*omegaR^2*vx*wn*wz*sign(omegaL) + 3.3e118*c21*omegaL^2*omegaR*vx*wn*wz*sign(omegaR) - 3.3e118*c12*omegaL*omegaR^2*vz*wn*wz*sign(omegaL) + 3.3e118*c12*omegaL^2*omegaR*vz*wn*wz*sign(omegaR) - 1.19e121*deltaL*omegaL*vx^2*vy*wn*sign(vx)*(vx^2 + vy^2)^(1/2) + 1.19e121*deltaR*omegaR*vx^2*vy*wn*sign(vx)*(vx^2 + vy^2)^(1/2) - 1.19e121*deltaL*omegaL*vy*vz^2*wn*sign(vx)*(vx^2 + vy^2)^(1/2) + 1.19e121*deltaR*omegaR*vy*vz^2*wn*sign(vx)*(vx^2 + vy^2)^(1/2) - 3.3e118*c22*omegaL^3*vx*vz*wn*wz*sign(omegaL) + 3.3e118*c22*omegaR^3*vx*vz*wn*wz*sign(omegaR) + 5.26e119*vx^2*vy*wn*cos(2.0*atan2(1.0*vy, vx))*abs(omegaL)*sign(vx)*(vx^2 + vy^2)^(1/2) - 5.26e119*vx^2*vy*wn*cos(2.0*atan2(1.0*vy, vx))*abs(omegaR)*sign(vx)*(vx^2 + vy^2)^(1/2) + 5.26e119*vy*vz^2*wn*cos(2.0*atan2(1.0*vy, vx))*abs(omegaL)*sign(vx)*(vx^2 + vy^2)^(1/2) - 5.26e119*vy*vz^2*wn*cos(2.0*atan2(1.0*vy, vx))*abs(omegaR)*sign(vx)*(vx^2 + vy^2)^(1/2) - 1.85e120*a33*omegaL*omegaR^2*vx^2*vz^2*wn*wx + 1.85e120*a33*omegaL^2*omegaR*vx^2*vz^2*wn*wx - 1.85e120*a43*omegaL*omegaR^2*vx^3*vz^2*wn*wx + 1.85e120*a43*omegaL^2*omegaR*vx^3*vz^2*wn*wx - 1.85e120*b33*omegaL*omegaR^2*vx^2*vz^2*wn*wz + 1.85e120*b33*omegaL^2*omegaR*vx^2*vz^2*wn*wz - 1.85e120*b34*omegaL*omegaR^2*vx^2*vz^3*wn*wz + 1.85e120*b34*omegaL^2*omegaR*vx^2*vz^3*wn*wz - 3.3e118*c23*omegaL^2*vx*vz^2*wn*wz*abs(omegaL) - 3.3e118*c24*omegaL^2*vx*vz^3*wn*wz*abs(omegaL) + 3.3e118*c23*omegaL^2*vx*vz^2*wn*wz*abs(omegaR) - 3.3e118*c23*omegaR^2*vx*vz^2*wn*wz*abs(omegaL) + 3.3e118*c24*omegaL^2*vx*vz^3*wn*wz*abs(omegaR) - 3.3e118*c24*omegaR^2*vx*vz^3*wn*wz*abs(omegaL) - 3.3e118*c32*omegaL^2*vx^2*vz*wn*wz*abs(omegaL) + 3.3e118*c23*omegaR^2*vx*vz^2*wn*wz*abs(omegaR) + 3.3e118*c24*omegaR^2*vx*vz^3*wn*wz*abs(omegaR) + 3.3e118*c32*omegaL^2*vx^2*vz*wn*wz*abs(omegaR) - 3.3e118*c32*omegaR^2*vx^2*vz*wn*wz*abs(omegaL) - 3.3e118*c42*omegaL^2*vx^3*vz*wn*wz*abs(omegaL) + 3.3e118*c32*omegaR^2*vx^2*vz*wn*wz*abs(omegaR) + 3.3e118*c42*omegaL^2*vx^3*vz*wn*wz*abs(omegaR) - 3.3e118*c42*omegaR^2*vx^3*vz*wn*wz*abs(omegaL) + 3.3e118*c42*omegaR^2*vx^3*vz*wn*wz*abs(omegaR) + 5.26e119*omegaL*vy^3*wn*cos(2.0*atan2(1.0*vy, vx))*sign(omegaL)*sign(vx)*(vx^2 + vy^2)^(1/2) - 5.26e119*omegaR*vy^3*wn*cos(2.0*atan2(1.0*vy, vx))*sign(omegaR)*sign(vx)*(vx^2 + vy^2)^(1/2) - 3.3e118*c31*omegaL*omegaR^2*vx^2*wn*wz*sign(omegaL) + 3.3e118*c31*omegaL^2*omegaR*vx^2*wn*wz*sign(omegaR) - 3.3e118*c41*omegaL*omegaR^2*vx^3*wn*wz*sign(omegaL) + 3.3e118*c41*omegaL^2*omegaR*vx^3*wn*wz*sign(omegaR) - 3.3e118*c13*omegaL*omegaR^2*vz^2*wn*wz*sign(omegaL) - 3.3e118*c14*omegaL*omegaR^2*vz^3*wn*wz*sign(omegaL) + 3.3e118*c13*omegaL^2*omegaR*vz^2*wn*wz*sign(omegaR) + 3.3e118*c14*omegaL^2*omegaR*vz^3*wn*wz*sign(omegaR) - 3.16e119*vx*vy^2*wn*sin(2.0*atan2(1.0*vy, vx))*abs(omegaL)*sign(vx)*(vx^2 + vy^2)^(1/2) + 3.16e119*vx*vy^2*wn*sin(2.0*atan2(1.0*vy, vx))*abs(omegaR)*sign(vx)*(vx^2 + vy^2)^(1/2) - 3.16e119*vx*vz^2*wn*sin(2.0*atan2(1.0*vy, vx))*abs(omegaL)*sign(vx)*(vx^2 + vy^2)^(1/2) + 3.16e119*vx*vz^2*wn*sin(2.0*atan2(1.0*vy, vx))*abs(omegaR)*sign(vx)*(vx^2 + vy^2)^(1/2) + 1.37e118*deltaL*omegaL*omegaR^2*vy*wn*cos(2.0*atan2(1.0*vy, vx))*(vx^2 + vy^2)^(1/2) - 1.37e118*deltaR*omegaL^2*omegaR*vy*wn*cos(2.0*atan2(1.0*vy, vx))*(vx^2 + vy^2)^(1/2) - 3.3e118*c23*omegaL^3*vx*vz^2*wn*wz*sign(omegaL) - 3.3e118*c24*omegaL^3*vx*vz^3*wn*wz*sign(omegaL) - 3.3e118*c32*omegaL^3*vx^2*vz*wn*wz*sign(omegaL) + 3.3e118*c23*omegaR^3*vx*vz^2*wn*wz*sign(omegaR) + 3.3e118*c24*omegaR^3*vx*vz^3*wn*wz*sign(omegaR) - 3.3e118*c42*omegaL^3*vx^3*vz*wn*wz*sign(omegaL) + 3.3e118*c32*omegaR^3*vx^2*vz*wn*wz*sign(omegaR) + 3.3e118*c42*omegaR^3*vx^3*vz*wn*wz*sign(omegaR) - 3.16e119*omegaL*vx^3*wn*sin(2.0*atan2(1.0*vy, vx))*sign(omegaL)*sign(vx)*(vx^2 + vy^2)^(1/2) + 3.16e119*omegaR*vx^3*wn*sin(2.0*atan2(1.0*vy, vx))*sign(omegaR)*sign(vx)*(vx^2 + vy^2)^(1/2) - 5.74e121*c21*vx*vy^2*wn*wz*abs(omegaL)*sign(vx) + 5.74e121*c21*vx*vy^2*wn*wz*abs(omegaR)*sign(vx) - 5.74e121*c12*vx^2*vz*wn*wz*abs(omegaL)*sign(vx) + 5.74e121*c12*vx^2*vz*wn*wz*abs(omegaR)*sign(vx) - 5.74e121*c21*vx*vz^2*wn*wz*abs(omegaL)*sign(vx) - 5.74e121*c22*vx*vz^3*wn*wz*abs(omegaL)*sign(vx) - 5.74e121*c22*vx^3*vz*wn*wz*abs(omegaL)*sign(vx) - 5.74e121*c23*vx*vz^4*wn*wz*abs(omegaL)*sign(vx) + 5.74e121*c21*vx*vz^2*wn*wz*abs(omegaR)*sign(vx) - 5.74e121*c24*vx*vz^5*wn*wz*abs(omegaL)*sign(vx) + 5.74e121*c22*vx*vz^3*wn*wz*abs(omegaR)*sign(vx) + 5.74e121*c22*vx^3*vz*wn*wz*abs(omegaR)*sign(vx) + 5.74e121*c23*vx*vz^4*wn*wz*abs(omegaR)*sign(vx) + 5.74e121*c24*vx*vz^5*wn*wz*abs(omegaR)*sign(vx) - 5.74e121*c32*vx^4*vz*wn*wz*abs(omegaL)*sign(vx) + 5.74e121*c32*vx^4*vz*wn*wz*abs(omegaR)*sign(vx) - 5.74e121*c42*vx^5*vz*wn*wz*abs(omegaL)*sign(vx) + 5.74e121*c42*vx^5*vz*wn*wz*abs(omegaR)*sign(vx) - 5.74e121*c12*vy^2*vz*wn*wz*abs(omegaL)*sign(vx) + 5.74e121*c12*vy^2*vz*wn*wz*abs(omegaR)*sign(vx) - 8.22e117*deltaL*omegaL*omegaR^2*vx*wn*sin(2.0*atan2(1.0*vy, vx))*(vx^2 + vy^2)^(1/2) + 8.22e117*deltaR*omegaL^2*omegaR*vx*wn*sin(2.0*atan2(1.0*vy, vx))*(vx^2 + vy^2)^(1/2) - 5.74e121*c11*omegaL*vx^2*wn*wz*sign(omegaL)*sign(vx) - 5.74e121*c21*omegaL*vx^3*wn*wz*sign(omegaL)*sign(vx) + 5.74e121*c11*omegaR*vx^2*wn*wz*sign(omegaR)*sign(vx) - 5.74e121*c31*omegaL*vx^4*wn*wz*sign(omegaL)*sign(vx) + 5.74e121*c21*omegaR*vx^3*wn*wz*sign(omegaR)*sign(vx) - 5.74e121*c41*omegaL*vx^5*wn*wz*sign(omegaL)*sign(vx) + 5.74e121*c31*omegaR*vx^4*wn*wz*sign(omegaR)*sign(vx) + 5.74e121*c41*omegaR*vx^5*wn*wz*sign(omegaR)*sign(vx) - 5.74e121*c11*omegaL*vy^2*wn*wz*sign(omegaL)*sign(vx) + 5.74e121*c11*omegaR*vy^2*wn*wz*sign(omegaR)*sign(vx) - 5.74e121*c11*omegaL*vz^2*wn*wz*sign(omegaL)*sign(vx) - 5.74e121*c12*omegaL*vz^3*wn*wz*sign(omegaL)*sign(vx) - 5.74e121*c13*omegaL*vz^4*wn*wz*sign(omegaL)*sign(vx) - 5.74e121*c14*omegaL*vz^5*wn*wz*sign(omegaL)*sign(vx) + 5.74e121*c11*omegaR*vz^2*wn*wz*sign(omegaR)*sign(vx) + 5.74e121*c12*omegaR*vz^3*wn*wz*sign(omegaR)*sign(vx) + 5.74e121*c13*omegaR*vz^4*wn*wz*sign(omegaR)*sign(vx) + 5.74e121*c14*omegaR*vz^5*wn*wz*sign(omegaR)*sign(vx) - 5.26e119*omegaL*vx^2*vy*wn*sign(omegaL)*sign(vx)*(vx^2 + vy^2)^(1/2) + 5.26e119*omegaR*vx^2*vy*wn*sign(omegaR)*sign(vx)*(vx^2 + vy^2)^(1/2) - 5.26e119*omegaL*vy*vz^2*wn*sign(omegaL)*sign(vx)*(vx^2 + vy^2)^(1/2) + 5.26e119*omegaR*vy*vz^2*wn*sign(omegaR)*sign(vx)*(vx^2 + vy^2)^(1/2) - 1.49e120*c21*deltaL*omegaL*omegaR^2*vx*wn*wz + 1.49e120*c21*deltaR*omegaL^2*omegaR*vx*wn*wz - 1.49e120*c12*deltaL*omegaL*omegaR^2*vz*wn*wz + 1.49e120*c12*deltaR*omegaL^2*omegaR*vz*wn*wz - 1.85e120*a22*omegaL*omegaR^2*vx*vz*wn*wx + 1.85e120*a22*omegaL^2*omegaR*vx*vz*wn*wx - 1.85e120*b22*omegaL*omegaR^2*vx*vz*wn*wz + 1.85e120*b22*omegaL^2*omegaR*vx*vz*wn*wz - 3.3e118*c33*omegaL^2*vx^2*vz^2*wn*wz*abs(omegaL) - 3.3e118*c34*omegaL^2*vx^2*vz^3*wn*wz*abs(omegaL) + 3.3e118*c33*omegaL^2*vx^2*vz^2*wn*wz*abs(omegaR) - 3.3e118*c33*omegaR^2*vx^2*vz^2*wn*wz*abs(omegaL) + 3.3e118*c34*omegaL^2*vx^2*vz^3*wn*wz*abs(omegaR) - 3.3e118*c34*omegaR^2*vx^2*vz^3*wn*wz*abs(omegaL) - 3.3e118*c43*omegaL^2*vx^3*vz^2*wn*wz*abs(omegaL) + 3.3e118*c33*omegaR^2*vx^2*vz^2*wn*wz*abs(omegaR) - 3.3e118*c44*omegaL^2*vx^3*vz^3*wn*wz*abs(omegaL) + 3.3e118*c34*omegaR^2*vx^2*vz^3*wn*wz*abs(omegaR) + 3.3e118*c43*omegaL^2*vx^3*vz^2*wn*wz*abs(omegaR) - 3.3e118*c43*omegaR^2*vx^3*vz^2*wn*wz*abs(omegaL) + 3.3e118*c44*omegaL^2*vx^3*vz^3*wn*wz*abs(omegaR) - 3.3e118*c44*omegaR^2*vx^3*vz^3*wn*wz*abs(omegaL) + 3.3e118*c43*omegaR^2*vx^3*vz^2*wn*wz*abs(omegaR) + 3.3e118*c44*omegaR^2*vx^3*vz^3*wn*wz*abs(omegaR) + 5.26e119*omegaL*vx^2*vy*wn*cos(2.0*atan2(1.0*vy, vx))*sign(omegaL)*sign(vx)*(vx^2 + vy^2)^(1/2) - 5.26e119*omegaR*vx^2*vy*wn*cos(2.0*atan2(1.0*vy, vx))*sign(omegaR)*sign(vx)*(vx^2 + vy^2)^(1/2) + 5.26e119*omegaL*vy*vz^2*wn*cos(2.0*atan2(1.0*vy, vx))*sign(omegaL)*sign(vx)*(vx^2 + vy^2)^(1/2) - 5.26e119*omegaR*vy*vz^2*wn*cos(2.0*atan2(1.0*vy, vx))*sign(omegaR)*sign(vx)*(vx^2 + vy^2)^(1/2) - 1.3e123*c31*deltaL*omegaL*vx^2*vy^2*wn*wz*sign(vx) - 1.3e123*c41*deltaL*omegaL*vx^3*vy^2*wn*wz*sign(vx) + 1.3e123*c31*deltaR*omegaR*vx^2*vy^2*wn*wz*sign(vx) + 1.3e123*c41*deltaR*omegaR*vx^3*vy^2*wn*wz*sign(vx) - 1.3e123*c13*deltaL*omegaL*vx^2*vz^2*wn*wz*sign(vx) - 1.3e123*c14*deltaL*omegaL*vx^2*vz^3*wn*wz*sign(vx) - 1.3e123*c23*deltaL*omegaL*vx^3*vz^2*wn*wz*sign(vx) + 1.3e123*c13*deltaR*omegaR*vx^2*vz^2*wn*wz*sign(vx) - 1.3e123*c24*deltaL*omegaL*vx^3*vz^3*wn*wz*sign(vx) + 1.3e123*c14*deltaR*omegaR*vx^2*vz^3*wn*wz*sign(vx) - 1.3e123*c31*deltaL*omegaL*vx^2*vz^2*wn*wz*sign(vx) - 1.3e123*c32*deltaL*omegaL*vx^2*vz^3*wn*wz*sign(vx) - 1.3e123*c33*deltaL*omegaL*vx^2*vz^4*wn*wz*sign(vx) - 1.3e123*c33*deltaL*omegaL*vx^4*vz^2*wn*wz*sign(vx) + 1.3e123*c23*deltaR*omegaR*vx^3*vz^2*wn*wz*sign(vx) - 1.3e123*c34*deltaL*omegaL*vx^2*vz^5*wn*wz*sign(vx) - 1.3e123*c34*deltaL*omegaL*vx^4*vz^3*wn*wz*sign(vx) + 1.3e123*c24*deltaR*omegaR*vx^3*vz^3*wn*wz*sign(vx) - 1.3e123*c41*deltaL*omegaL*vx^3*vz^2*wn*wz*sign(vx) + 1.3e123*c31*deltaR*omegaR*vx^2*vz^2*wn*wz*sign(vx) - 1.3e123*c42*deltaL*omegaL*vx^3*vz^3*wn*wz*sign(vx) + 1.3e123*c32*deltaR*omegaR*vx^2*vz^3*wn*wz*sign(vx) - 1.3e123*c43*deltaL*omegaL*vx^3*vz^4*wn*wz*sign(vx) - 1.3e123*c43*deltaL*omegaL*vx^5*vz^2*wn*wz*sign(vx) + 1.3e123*c33*deltaR*omegaR*vx^2*vz^4*wn*wz*sign(vx) + 1.3e123*c33*deltaR*omegaR*vx^4*vz^2*wn*wz*sign(vx) - 1.3e123*c44*deltaL*omegaL*vx^3*vz^5*wn*wz*sign(vx) - 1.3e123*c44*deltaL*omegaL*vx^5*vz^3*wn*wz*sign(vx) + 1.3e123*c34*deltaR*omegaR*vx^2*vz^5*wn*wz*sign(vx) + 1.3e123*c34*deltaR*omegaR*vx^4*vz^3*wn*wz*sign(vx) + 1.3e123*c41*deltaR*omegaR*vx^3*vz^2*wn*wz*sign(vx) + 1.3e123*c42*deltaR*omegaR*vx^3*vz^3*wn*wz*sign(vx) + 1.3e123*c43*deltaR*omegaR*vx^3*vz^4*wn*wz*sign(vx) + 1.3e123*c43*deltaR*omegaR*vx^5*vz^2*wn*wz*sign(vx) + 1.3e123*c44*deltaR*omegaR*vx^3*vz^5*wn*wz*sign(vx) + 1.3e123*c44*deltaR*omegaR*vx^5*vz^3*wn*wz*sign(vx) - 1.3e123*c13*deltaL*omegaL*vy^2*vz^2*wn*wz*sign(vx) - 1.3e123*c14*deltaL*omegaL*vy^2*vz^3*wn*wz*sign(vx) + 1.3e123*c13*deltaR*omegaR*vy^2*vz^2*wn*wz*sign(vx) + 1.3e123*c14*deltaR*omegaR*vy^2*vz^3*wn*wz*sign(vx) - 3.3e118*c23*omegaL*omegaR^2*vx*vz^2*wn*wz*sign(omegaL) - 3.3e118*c24*omegaL*omegaR^2*vx*vz^3*wn*wz*sign(omegaL) + 3.3e118*c23*omegaL^2*omegaR*vx*vz^2*wn*wz*sign(omegaR) + 3.3e118*c24*omegaL^2*omegaR*vx*vz^3*wn*wz*sign(omegaR) - 3.3e118*c32*omegaL*omegaR^2*vx^2*vz*wn*wz*sign(omegaL) + 3.3e118*c32*omegaL^2*omegaR*vx^2*vz*wn*wz*sign(omegaR) - 3.3e118*c42*omegaL*omegaR^2*vx^3*vz*wn*wz*sign(omegaL) + 3.3e118*c42*omegaL^2*omegaR*vx^3*vz*wn*wz*sign(omegaR) - 3.16e119*omegaL*vx*vy^2*wn*sin(2.0*atan2(1.0*vy, vx))*sign(omegaL)*sign(vx)*(vx^2 + vy^2)^(1/2) + 3.16e119*omegaR*vx*vy^2*wn*sin(2.0*atan2(1.0*vy, vx))*sign(omegaR)*sign(vx)*(vx^2 + vy^2)^(1/2) - 3.16e119*omegaL*vx*vz^2*wn*sin(2.0*atan2(1.0*vy, vx))*sign(omegaL)*sign(vx)*(vx^2 + vy^2)^(1/2) + 3.16e119*omegaR*vx*vz^2*wn*sin(2.0*atan2(1.0*vy, vx))*sign(omegaR)*sign(vx)*(vx^2 + vy^2)^(1/2) - 5.74e121*c22*vx*vy^2*vz*wn*wz*abs(omegaL)*sign(vx) + 5.74e121*c22*vx*vy^2*vz*wn*wz*abs(omegaR)*sign(vx) - 5.74e121*c21*omegaL*vx*vy^2*wn*wz*sign(omegaL)*sign(vx) + 5.74e121*c21*omegaR*vx*vy^2*wn*wz*sign(omegaR)*sign(vx) - 5.74e121*c12*omegaL*vx^2*vz*wn*wz*sign(omegaL)*sign(vx) - 5.74e121*c21*omegaL*vx*vz^2*wn*wz*sign(omegaL)*sign(vx) - 5.74e121*c22*omegaL*vx*vz^3*wn*wz*sign(omegaL)*sign(vx) - 5.74e121*c22*omegaL*vx^3*vz*wn*wz*sign(omegaL)*sign(vx) + 5.74e121*c12*omegaR*vx^2*vz*wn*wz*sign(omegaR)*sign(vx) - 5.74e121*c23*omegaL*vx*vz^4*wn*wz*sign(omegaL)*sign(vx) - 5.74e121*c24*omegaL*vx*vz^5*wn*wz*sign(omegaL)*sign(vx) + 5.74e121*c21*omegaR*vx*vz^2*wn*wz*sign(omegaR)*sign(vx) - 5.74e121*c32*omegaL*vx^4*vz*wn*wz*sign(omegaL)*sign(vx) + 5.74e121*c22*omegaR*vx*vz^3*wn*wz*sign(omegaR)*sign(vx) + 5.74e121*c22*omegaR*vx^3*vz*wn*wz*sign(omegaR)*sign(vx) + 5.74e121*c23*omegaR*vx*vz^4*wn*wz*sign(omegaR)*sign(vx) + 5.74e121*c24*omegaR*vx*vz^5*wn*wz*sign(omegaR)*sign(vx) - 5.74e121*c42*omegaL*vx^5*vz*wn*wz*sign(omegaL)*sign(vx) + 5.74e121*c32*omegaR*vx^4*vz*wn*wz*sign(omegaR)*sign(vx) + 5.74e121*c42*omegaR*vx^5*vz*wn*wz*sign(omegaR)*sign(vx) - 5.74e121*c12*omegaL*vy^2*vz*wn*wz*sign(omegaL)*sign(vx) + 5.74e121*c12*omegaR*vy^2*vz*wn*wz*sign(omegaR)*sign(vx) - 1.49e120*c22*deltaL*omegaL*omegaR^2*vx*vz*wn*wz + 1.49e120*c22*deltaR*omegaL^2*omegaR*vx*vz*wn*wz - 3.3e118*c33*omegaL*omegaR^2*vx^2*vz^2*wn*wz*sign(omegaL) - 3.3e118*c34*omegaL*omegaR^2*vx^2*vz^3*wn*wz*sign(omegaL) + 3.3e118*c33*omegaL^2*omegaR*vx^2*vz^2*wn*wz*sign(omegaR) + 3.3e118*c34*omegaL^2*omegaR*vx^2*vz^3*wn*wz*sign(omegaR) - 3.3e118*c43*omegaL*omegaR^2*vx^3*vz^2*wn*wz*sign(omegaL) - 3.3e118*c44*omegaL*omegaR^2*vx^3*vz^3*wn*wz*sign(omegaL) + 3.3e118*c43*omegaL^2*omegaR*vx^3*vz^2*wn*wz*sign(omegaR) + 3.3e118*c44*omegaL^2*omegaR*vx^3*vz^3*wn*wz*sign(omegaR) - 5.74e121*c23*vx*vy^2*vz^2*wn*wz*abs(omegaL)*sign(vx) - 5.74e121*c24*vx*vy^2*vz^3*wn*wz*abs(omegaL)*sign(vx) + 5.74e121*c23*vx*vy^2*vz^2*wn*wz*abs(omegaR)*sign(vx) + 5.74e121*c24*vx*vy^2*vz^3*wn*wz*abs(omegaR)*sign(vx) - 5.74e121*c32*vx^2*vy^2*vz*wn*wz*abs(omegaL)*sign(vx) + 5.74e121*c32*vx^2*vy^2*vz*wn*wz*abs(omegaR)*sign(vx) - 5.74e121*c42*vx^3*vy^2*vz*wn*wz*abs(omegaL)*sign(vx) + 5.74e121*c42*vx^3*vy^2*vz*wn*wz*abs(omegaR)*sign(vx) - 5.74e121*c31*omegaL*vx^2*vy^2*wn*wz*sign(omegaL)*sign(vx) - 5.74e121*c41*omegaL*vx^3*vy^2*wn*wz*sign(omegaL)*sign(vx) + 5.74e121*c31*omegaR*vx^2*vy^2*wn*wz*sign(omegaR)*sign(vx) + 5.74e121*c41*omegaR*vx^3*vy^2*wn*wz*sign(omegaR)*sign(vx) - 5.74e121*c13*omegaL*vx^2*vz^2*wn*wz*sign(omegaL)*sign(vx) - 5.74e121*c14*omegaL*vx^2*vz^3*wn*wz*sign(omegaL)*sign(vx) - 5.74e121*c23*omegaL*vx^3*vz^2*wn*wz*sign(omegaL)*sign(vx) + 5.74e121*c13*omegaR*vx^2*vz^2*wn*wz*sign(omegaR)*sign(vx) - 5.74e121*c24*omegaL*vx^3*vz^3*wn*wz*sign(omegaL)*sign(vx) + 5.74e121*c14*omegaR*vx^2*vz^3*wn*wz*sign(omegaR)*sign(vx) - 5.74e121*c31*omegaL*vx^2*vz^2*wn*wz*sign(omegaL)*sign(vx) - 5.74e121*c32*omegaL*vx^2*vz^3*wn*wz*sign(omegaL)*sign(vx) - 5.74e121*c33*omegaL*vx^2*vz^4*wn*wz*sign(omegaL)*sign(vx) - 5.74e121*c33*omegaL*vx^4*vz^2*wn*wz*sign(omegaL)*sign(vx) + 5.74e121*c23*omegaR*vx^3*vz^2*wn*wz*sign(omegaR)*sign(vx) - 5.74e121*c34*omegaL*vx^2*vz^5*wn*wz*sign(omegaL)*sign(vx) - 5.74e121*c34*omegaL*vx^4*vz^3*wn*wz*sign(omegaL)*sign(vx) + 5.74e121*c24*omegaR*vx^3*vz^3*wn*wz*sign(omegaR)*sign(vx) - 5.74e121*c41*omegaL*vx^3*vz^2*wn*wz*sign(omegaL)*sign(vx) + 5.74e121*c31*omegaR*vx^2*vz^2*wn*wz*sign(omegaR)*sign(vx) - 5.74e121*c42*omegaL*vx^3*vz^3*wn*wz*sign(omegaL)*sign(vx) + 5.74e121*c32*omegaR*vx^2*vz^3*wn*wz*sign(omegaR)*sign(vx) - 5.74e121*c43*omegaL*vx^3*vz^4*wn*wz*sign(omegaL)*sign(vx) - 5.74e121*c43*omegaL*vx^5*vz^2*wn*wz*sign(omegaL)*sign(vx) + 5.74e121*c33*omegaR*vx^2*vz^4*wn*wz*sign(omegaR)*sign(vx) + 5.74e121*c33*omegaR*vx^4*vz^2*wn*wz*sign(omegaR)*sign(vx) - 5.74e121*c44*omegaL*vx^3*vz^5*wn*wz*sign(omegaL)*sign(vx) - 5.74e121*c44*omegaL*vx^5*vz^3*wn*wz*sign(omegaL)*sign(vx) + 5.74e121*c34*omegaR*vx^2*vz^5*wn*wz*sign(omegaR)*sign(vx) + 5.74e121*c34*omegaR*vx^4*vz^3*wn*wz*sign(omegaR)*sign(vx) + 5.74e121*c41*omegaR*vx^3*vz^2*wn*wz*sign(omegaR)*sign(vx) + 5.74e121*c42*omegaR*vx^3*vz^3*wn*wz*sign(omegaR)*sign(vx) + 5.74e121*c43*omegaR*vx^3*vz^4*wn*wz*sign(omegaR)*sign(vx) + 5.74e121*c43*omegaR*vx^5*vz^2*wn*wz*sign(omegaR)*sign(vx) + 5.74e121*c44*omegaR*vx^3*vz^5*wn*wz*sign(omegaR)*sign(vx) + 5.74e121*c44*omegaR*vx^5*vz^3*wn*wz*sign(omegaR)*sign(vx) - 5.74e121*c13*omegaL*vy^2*vz^2*wn*wz*sign(omegaL)*sign(vx) - 5.74e121*c14*omegaL*vy^2*vz^3*wn*wz*sign(omegaL)*sign(vx) + 5.74e121*c13*omegaR*vy^2*vz^2*wn*wz*sign(omegaR)*sign(vx) + 5.74e121*c14*omegaR*vy^2*vz^3*wn*wz*sign(omegaR)*sign(vx) + 1.19e121*deltaL*omegaL*vx^2*vy*wn*cos(2.0*atan2(1.0*vy, vx))*sign(vx)*(vx^2 + vy^2)^(1/2) - 1.19e121*deltaR*omegaR*vx^2*vy*wn*cos(2.0*atan2(1.0*vy, vx))*sign(vx)*(vx^2 + vy^2)^(1/2) + 1.19e121*deltaL*omegaL*vy*vz^2*wn*cos(2.0*atan2(1.0*vy, vx))*sign(vx)*(vx^2 + vy^2)^(1/2) - 1.19e121*deltaR*omegaR*vy*vz^2*wn*cos(2.0*atan2(1.0*vy, vx))*sign(vx)*(vx^2 + vy^2)^(1/2) - 1.49e120*c23*deltaL*omegaL*omegaR^2*vx*vz^2*wn*wz - 1.49e120*c24*deltaL*omegaL*omegaR^2*vx*vz^3*wn*wz + 1.49e120*c23*deltaR*omegaL^2*omegaR*vx*vz^2*wn*wz + 1.49e120*c24*deltaR*omegaL^2*omegaR*vx*vz^3*wn*wz - 1.49e120*c32*deltaL*omegaL*omegaR^2*vx^2*vz*wn*wz + 1.49e120*c32*deltaR*omegaL^2*omegaR*vx^2*vz*wn*wz - 1.49e120*c42*deltaL*omegaL*omegaR^2*vx^3*vz*wn*wz + 1.49e120*c42*deltaR*omegaL^2*omegaR*vx^3*vz*wn*wz - 7.14e120*deltaL*omegaL*vx*vy^2*wn*sin(2.0*atan2(1.0*vy, vx))*sign(vx)*(vx^2 + vy^2)^(1/2) + 7.14e120*deltaR*omegaR*vx*vy^2*wn*sin(2.0*atan2(1.0*vy, vx))*sign(vx)*(vx^2 + vy^2)^(1/2) - 7.14e120*deltaL*omegaL*vx*vz^2*wn*sin(2.0*atan2(1.0*vy, vx))*sign(vx)*(vx^2 + vy^2)^(1/2) + 7.14e120*deltaR*omegaR*vx*vz^2*wn*sin(2.0*atan2(1.0*vy, vx))*sign(vx)*(vx^2 + vy^2)^(1/2) - 1.3e123*c21*deltaL*omegaL*vx*vy^2*wn*wz*sign(vx) + 1.3e123*c21*deltaR*omegaR*vx*vy^2*wn*wz*sign(vx) - 1.3e123*c12*deltaL*omegaL*vx^2*vz*wn*wz*sign(vx) - 1.3e123*c21*deltaL*omegaL*vx*vz^2*wn*wz*sign(vx) - 1.3e123*c22*deltaL*omegaL*vx*vz^3*wn*wz*sign(vx) - 1.3e123*c22*deltaL*omegaL*vx^3*vz*wn*wz*sign(vx) + 1.3e123*c12*deltaR*omegaR*vx^2*vz*wn*wz*sign(vx) - 1.3e123*c23*deltaL*omegaL*vx*vz^4*wn*wz*sign(vx) - 1.3e123*c24*deltaL*omegaL*vx*vz^5*wn*wz*sign(vx) + 1.3e123*c21*deltaR*omegaR*vx*vz^2*wn*wz*sign(vx) - 1.3e123*c32*deltaL*omegaL*vx^4*vz*wn*wz*sign(vx) + 1.3e123*c22*deltaR*omegaR*vx*vz^3*wn*wz*sign(vx) + 1.3e123*c22*deltaR*omegaR*vx^3*vz*wn*wz*sign(vx) + 1.3e123*c23*deltaR*omegaR*vx*vz^4*wn*wz*sign(vx) + 1.3e123*c24*deltaR*omegaR*vx*vz^5*wn*wz*sign(vx) - 1.3e123*c42*deltaL*omegaL*vx^5*vz*wn*wz*sign(vx) + 1.3e123*c32*deltaR*omegaR*vx^4*vz*wn*wz*sign(vx) + 1.3e123*c42*deltaR*omegaR*vx^5*vz*wn*wz*sign(vx) - 1.3e123*c12*deltaL*omegaL*vy^2*vz*wn*wz*sign(vx) + 1.3e123*c12*deltaR*omegaR*vy^2*vz*wn*wz*sign(vx) - 3.3e118*c22*omegaL*omegaR^2*vx*vz*wn*wz*sign(omegaL) + 3.3e118*c22*omegaL^2*omegaR*vx*vz*wn*wz*sign(omegaR) - 5.74e121*c33*vx^2*vy^2*vz^2*wn*wz*abs(omegaL)*sign(vx) - 5.74e121*c34*vx^2*vy^2*vz^3*wn*wz*abs(omegaL)*sign(vx) + 5.74e121*c33*vx^2*vy^2*vz^2*wn*wz*abs(omegaR)*sign(vx) + 5.74e121*c34*vx^2*vy^2*vz^3*wn*wz*abs(omegaR)*sign(vx) - 5.74e121*c43*vx^3*vy^2*vz^2*wn*wz*abs(omegaL)*sign(vx) - 5.74e121*c44*vx^3*vy^2*vz^3*wn*wz*abs(omegaL)*sign(vx) + 5.74e121*c43*vx^3*vy^2*vz^2*wn*wz*abs(omegaR)*sign(vx) + 5.74e121*c44*vx^3*vy^2*vz^3*wn*wz*abs(omegaR)*sign(vx) - 1.49e120*c33*deltaL*omegaL*omegaR^2*vx^2*vz^2*wn*wz - 1.49e120*c34*deltaL*omegaL*omegaR^2*vx^2*vz^3*wn*wz + 1.49e120*c33*deltaR*omegaL^2*omegaR*vx^2*vz^2*wn*wz + 1.49e120*c34*deltaR*omegaL^2*omegaR*vx^2*vz^3*wn*wz - 1.49e120*c43*deltaL*omegaL*omegaR^2*vx^3*vz^2*wn*wz - 1.49e120*c44*deltaL*omegaL*omegaR^2*vx^3*vz^3*wn*wz + 1.49e120*c43*deltaR*omegaL^2*omegaR*vx^3*vz^2*wn*wz + 1.49e120*c44*deltaR*omegaL^2*omegaR*vx^3*vz^3*wn*wz - 5.74e121*c23*omegaL*vx*vy^2*vz^2*wn*wz*sign(omegaL)*sign(vx) - 5.74e121*c24*omegaL*vx*vy^2*vz^3*wn*wz*sign(omegaL)*sign(vx) - 5.74e121*c32*omegaL*vx^2*vy^2*vz*wn*wz*sign(omegaL)*sign(vx) + 5.74e121*c23*omegaR*vx*vy^2*vz^2*wn*wz*sign(omegaR)*sign(vx) + 5.74e121*c24*omegaR*vx*vy^2*vz^3*wn*wz*sign(omegaR)*sign(vx) - 5.74e121*c42*omegaL*vx^3*vy^2*vz*wn*wz*sign(omegaL)*sign(vx) + 5.74e121*c32*omegaR*vx^2*vy^2*vz*wn*wz*sign(omegaR)*sign(vx) + 5.74e121*c42*omegaR*vx^3*vy^2*vz*wn*wz*sign(omegaR)*sign(vx) - 1.3e123*c22*deltaL*omegaL*vx*vy^2*vz*wn*wz*sign(vx) + 1.3e123*c22*deltaR*omegaR*vx*vy^2*vz*wn*wz*sign(vx) - 5.74e121*c33*omegaL*vx^2*vy^2*vz^2*wn*wz*sign(omegaL)*sign(vx) - 5.74e121*c34*omegaL*vx^2*vy^2*vz^3*wn*wz*sign(omegaL)*sign(vx) - 5.74e121*c43*omegaL*vx^3*vy^2*vz^2*wn*wz*sign(omegaL)*sign(vx) + 5.74e121*c33*omegaR*vx^2*vy^2*vz^2*wn*wz*sign(omegaR)*sign(vx) - 5.74e121*c44*omegaL*vx^3*vy^2*vz^3*wn*wz*sign(omegaL)*sign(vx) + 5.74e121*c34*omegaR*vx^2*vy^2*vz^3*wn*wz*sign(omegaR)*sign(vx) + 5.74e121*c43*omegaR*vx^3*vy^2*vz^2*wn*wz*sign(omegaR)*sign(vx) + 5.74e121*c44*omegaR*vx^3*vy^2*vz^3*wn*wz*sign(omegaR)*sign(vx) - 1.3e123*c23*deltaL*omegaL*vx*vy^2*vz^2*wn*wz*sign(vx) - 1.3e123*c24*deltaL*omegaL*vx*vy^2*vz^3*wn*wz*sign(vx) - 1.3e123*c32*deltaL*omegaL*vx^2*vy^2*vz*wn*wz*sign(vx) + 1.3e123*c23*deltaR*omegaR*vx*vy^2*vz^2*wn*wz*sign(vx) + 1.3e123*c24*deltaR*omegaR*vx*vy^2*vz^3*wn*wz*sign(vx) - 1.3e123*c42*deltaL*omegaL*vx^3*vy^2*vz*wn*wz*sign(vx) + 1.3e123*c32*deltaR*omegaR*vx^2*vy^2*vz*wn*wz*sign(vx) + 1.3e123*c42*deltaR*omegaR*vx^3*vy^2*vz*wn*wz*sign(vx) - 5.74e121*c22*omegaL*vx*vy^2*vz*wn*wz*sign(omegaL)*sign(vx) + 5.74e121*c22*omegaR*vx*vy^2*vz*wn*wz*sign(omegaR)*sign(vx) - 1.3e123*c33*deltaL*omegaL*vx^2*vy^2*vz^2*wn*wz*sign(vx) - 1.3e123*c34*deltaL*omegaL*vx^2*vy^2*vz^3*wn*wz*sign(vx) - 1.3e123*c43*deltaL*omegaL*vx^3*vy^2*vz^2*wn*wz*sign(vx) + 1.3e123*c33*deltaR*omegaR*vx^2*vy^2*vz^2*wn*wz*sign(vx) - 1.3e123*c44*deltaL*omegaL*vx^3*vy^2*vz^3*wn*wz*sign(vx) + 1.3e123*c34*deltaR*omegaR*vx^2*vy^2*vz^3*wn*wz*sign(vx) + 1.3e123*c43*deltaR*omegaR*vx^3*vy^2*vz^2*wn*wz*sign(vx) + 1.3e123*c44*deltaR*omegaR*vx^3*vy^2*vz^3*wn*wz*sign(vx)))/((omegaL + omegaR)*(2.9e93*omegaL^2*omegaR^2 + 2.52e96*omegaL^2*vx^2*sign(vx) + 2.52e96*omegaL^2*vy^2*sign(vx) + 2.52e96*omegaL^2*vz^2*sign(vx) + 2.52e96*omegaR^2*vx^2*sign(vx) + 2.52e96*omegaR^2*vy^2*sign(vx) + 2.52e96*omegaR^2*vz^2*sign(vx) + 2.19e99*vx^4*sign(vx)^2 + 4.37e99*vx^2*vy^2*sign(vx)^2 + 4.37e99*vx^2*vz^2*sign(vx)^2 + 2.19e99*vy^4*sign(vx)^2 + 4.37e99*vy^2*vz^2*sign(vx)^2 + 2.19e99*vz^4*sign(vx)^2));
